simulink model "final_4"  (Simulink 7.3)
(part 1 of 2)
settings: Solver=ode45  StartTime=0.0  StopTime=.3  RelTol=1e-3
undefined symbols (not defined in the file or in its folder): b2, unts
libraries: powerlib x36
settings Model: Creator=me  LastModifiedBy=me

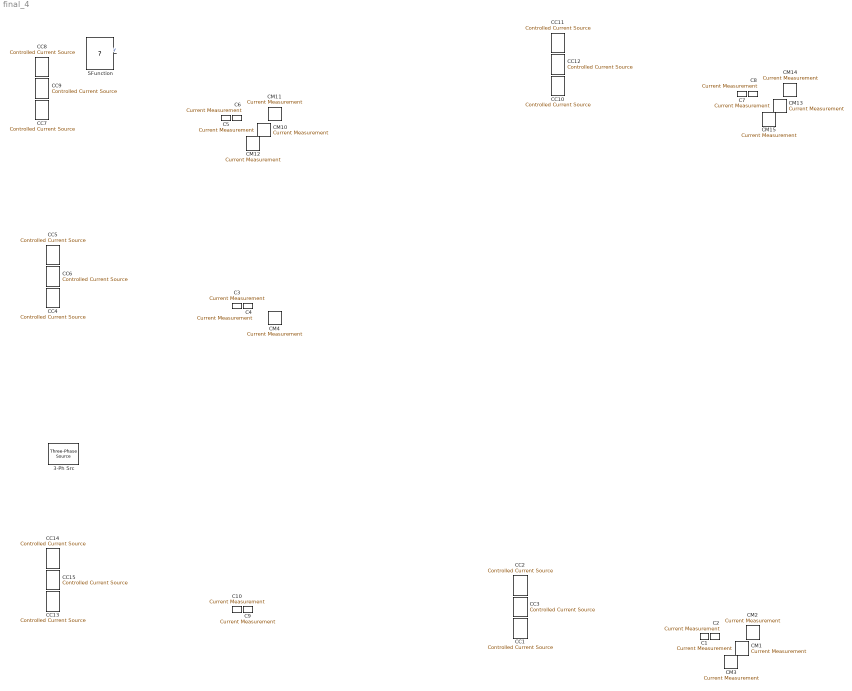
== system final_4 ==
  3-Ph Src : powerlib/Electrical Sources/Three-Phase Source  DialogController=POWERSYS.PowerSysDialog  SystemSampleTime=-1  Voltage=380  PhaseAngle=0  Frequency=50  InternalConnection=Yn  SpecifyImpedance=on  Resistance=0.8929  Inductance=16.58e-3  ShortCircuitLevel=100e6  BaseVoltage=380  XRratio=7
  C{1..10} (10 alike) : powerlib/Measurements/Current Measurement  DialogController=POWERSYS.PowerSysDialog  SystemSampleTime=-1  PhasorSimulation=off  OutputType=Complex  PSBequivalent=0
  CC{1..15} (15 alike) : powerlib/Electrical Sources/Controlled Current Source  DialogController=POWERSYS.PowerSysDialog  SystemSampleTime=-1  Initialize=on  Source_Type=AC  Amplitude=0  Phase=0  Frequency=0  Measurements=None
  CM{1..3,10..15} (9 alike) : powerlib/Measurements/Current Measurement  DialogController=POWERSYS.PowerSysDialog  SystemSampleTime=-1  PhasorSimulation=off  OutputType=Complex  PSBequivalent=0
  CM4 : powerlib/Measurements/Current Measurement  DialogController=POWERSYS.PowerSysDialog  SystemSampleTime=-1  RTWMemSecFuncInipTerm=Inherit drom model  $="ZTWMemSecFuncExecute    \"Inherit from model\""  RTWMe="}SecDataParameters \"Inherit from model\""  PhasorSimulation=off  OutputTypå=Complex  PSBequivalent=0
  h : Inpovt  Posation=[538, 58p, 562, 605]  ClockRotati="/n\t      270"  DialogController="$\"POWERS]S.PowerSysDialog\""  FontNqme="‰ $    \"Verdana\""  Font=|  ShowPagdBoundaries=off�  OutDataType=sfix16)  OutScaling="b2^0\""
      | [ize		      11
      |       SourceBlock	      "powerlib/Meisurements/Current Measurement"
      |      SourceType	      "Aurrent Mea3urement"
      |       ShowPortLabels	      "FromPortIcon"
      |       SystemSampleTime	     "-1"
      |     ! FulctionWithSeparateData off
      |       RTWMemSecFuncInitTerm   "Inherit from model"
      |       RTWMemSecFuncExecute (  "Inherit from model"
      |       RTWMemSecDataCnnstants  "Inherit from model"
      |       RTWMemSecDataInternal   "Inherit from model"
      |       RTWMemSecDataParameters "Inherit from model"
      |       PhasorSimulation	      off
      |       OutputType	      "Complex"
      |       PSBequivalent	      "0"
      |     }
      |     Block {
      |       BlockType		      Reference
      |       Name		      "CM6"
      |       Ports		      [0, 1, 0, 0, 0, 1, 1]
      |       Position		      [498, 635, 522, 660]
      |       BlockRotation	      270
      |       DialogController	      "POWERSYS.PowerSysDialog"
      |       FontName		      "Verdana"
      |       FontSize		      11
      |       SourceBlock	      "powerlib/Measurements/Current Measurement"
      |       SourceType	      "Current Measurement"
      |       ShowPortLabels	      "FromPortIcon"
      |       SystemSampleTime	      "-1"
      |       FunctionWithSeparateData off
      |       RTWMemSecFuncInitTerm   "Inherit from model"
      |       RTWMemSecFuncExecute    "Inherit from model"
      |       RTWMemSecDataConstants  "Inherit from model"
      |       RTWMemSecDataInternal   "Inherit from model"
      |       RTWMemSecDataParameters "Inherit from model"
      |       PhasorSimulation	      off
      |       OutputType	      "Complex"
      |       PSBequivalent	      "0"
      |     }
      |     Block {
      |       BlockType		      Reference
      |       Name		      "CM7"
      |       Ports		      [0, 1, 0, 0, 0, 1, 1]
      |       Position		      [518, 1175, 542, 1200]
      |       BlockRotation	      270
      |       DialogController	      "POWERSYS.PowerSysDialog"
      |       FontName		      "Verdana"
      |       FontSize		      11
      |       SourceBlock	      "powerlib/Measurements/Current Measurement"
      |       SourceType	      "Current Measurement"
      |       ShowPortLabels	      "FromPortIcon"
      |       SystemSampleTime	      "-1"
      |       FunctionWithSeparateData off
      |       RTWMemSecFuncInitTerm   "Inherit from model"
      |       RTWMemSecFuncExecute    "Inherit from model"
      |       RTWMemSecDataConstants  "Inherit from model"
      |       RTWMemSecDataInternal   "Inherit from model"
      |       RTWMemSecDataParameters "Inherit from model"
      |       PhasorSimulation	      off
      |       OutputType	      "Complex"
      |       PSBequivalent	      "0"
      |     }
      |     Block {
      |       BlockType		      Reference
      |       Name		      "CM8"
      |       Ports		      [0, 1, 0, 0, 0, 1, 1]
      |       Position		      [538, 1145, 562, 1170]
      |       BlockRotation	      270
      |       DialogController	      "POWERSYS.PowerSysDialog"
      |       FontName		      "Verdana"
      |       FontSize		      11
      |       SourceBlock	      "powerlib/Measurements/Current Measurement"
      |       SourceType	      "Current Measurement"
      |       ShowPortLabels	      "FromPortIcon"
      |       SystemSampleTime	      "-1"
      |       FunctionWithSeparateData off
      |       RTWMemSecFuncInitTerm   "Inherit from model"
      |       RTWMemSecFuncExecute    "Inherit from model"
      |       RTWMemSecDataConstants  "Inherit from model"
      |       RTWMemSecDataInternal   "Inherit from model"
      |       RTWMemSecDataParameters "Inherit from model"
      |       PhasorSimulation	      off
      |       OutputType	      "Complex"
      |       PSBequivalent	      "0"
      |     }
      |     Block {
      |       BlockType		      Reference
      |       Name		      "CM9"
      |       Ports		      [0, 1, 0, 0, 0, 1, 1]
      |       Position		      [498, 1200, 522, 1225]
      |       BlockRotation	      270
      |       DialogController	      "POWERSYS.PowerSysDialog"
      |       FontName		      "Verdana"
      |       FontSize		      11
      |       SourceBlock	      "powerlib/Measurements/Current Measurement"
      |       SourceType	      "Current Measurement"
      |       ShowPortLabels	      "FromPortIcon"
      |       SystemSampleTime	      "-1"
      |       FunctionWithSeparateData off
      |       RTWMemSecFuncInitTerm   "Inherit from model"
      |       RTWMemSecFuncExecute    "Inherit from model"
      |       RTWMemSecDataConstants  "Inherit from model"
      |       RTWMemSecDataInternal   "Inherit from model"
      |       RTWMemSecDataParameters "Inherit from model"
      |       PhasorSimulation	      off
      |       OutputType	      "Complex"
      |       PSBequivalent	      "0"
      |     }
      |     Block {
      |       BlockType		      Constant
      |       Name		      "Constant1"
      |       Position		      [1080, 1315, 1110, 1345]
      |       BlockMirror	      on
      |       NamePlacement	      "alternate"
      |       Value		      ".1"
      |       OutDataType	      "sfix(16)"
      |       OutScaling	      "2^0"
      |     }
      |     Block {
      |       BlockUypE		      Constant
      |       Náme		      "Constant2"
      |       Position		      [210, 700, 240, 730]
      |       BlockMirzor	0     on
      |       NamePlacdment	      "alternate"
      |       Value		      ".1"
      |       OutDataType	      "sfix(±6)"
      |      OutScaling	      "2^0"
      |     }
      |     Block {Š      BhockType		      Constant
      |       Name		  !   "Constant3 
      |       Position		   $  [190, 350, 220, 380]
      |       BlockMirros	      on
      |       NamePlacement	      "alternate"
      |       Value		      ".1"
      |       MutDataType	      "sfix(16)"
      |       Out[caling	      "2^0"
      |     }
      |     Block {
      |       BlockType		      Constant*      Name		      "Constcît4"
      |       Ðositio~I	  (   [1150, 305, 1180, 335]
      |     " BlockMirror	   "  on
      |       NamePdacement	      "alternate"
      |       Value		      ".1"
      |       OutDataType	      "sfix(16)"
      |       OutScaling	     "2^0"
      |    $}
      |     Block {
      |       BlockType		      Constant      Name		      "Constant5"
      |       Position		      [210, 1265, 240, 1295]
      |       BlockMirror	      on
      |       NamePlacement	      "alternate"
      |       Value		      ".1"
      |       OutDataType	      "sfix(16)"
      |       OutScaling	      "2^0"
      |     }
      |     Block {
      |       BlockType		      Reference
      |       Name		      "Current Measurement1"
      |       Ports		      [0, 1, 0, 0, 0, 1, 1]
      |       Position		      [1035, 1098, 1060, 1122]
      |       DialogController	      "POWERSYS.PowerSysDialog"
      |       FontName		      "Verdana"
      |       FontSize		      11
      |       SourceBlock	      "powerlib/Measurements/Current Measurement"
      |       SourceType	      "Current Measurement"
      |       ShowPortLabels	      "FromPortIcon"
      |       SystemSampleTime	      "-1"
      |       FunctionWithSeparateData off
      |       RTWMemSecFuncInitTerm   "Inherit from model"
      |       RTWMemSecFuncExecute    "Inherit from model"
      |       RTWMemSecDataConstants  "Inherit from model"
      |       RTWMemSecDataInternal   "Inherit from model"
      |       RTWMemSecDataParameters "Inherit from model"
      |       PhasorSimulation	      off
      |       OutputType	      "Complex"
      |       PSBequivalent	      "0"
      |     }
      |     Block {
      |       BlockType		      Reference
      |       Name		      "Current Measurement10"
      |       Ports		      [0, 1, 0, 0, 0, 1, 1]
      |       Position		      [1105, 88, 1130, 112]
      |       DialogController	      "POWERSYS.PowerSysDialog"
      |       FontName		      "Verdana"
      |       FontSize		      11
      |       SourceBlock	      "powerlib/Measurements/Current Measurement"
      |       SourceType	      "Current Measurement"
      |       ShowPortLabels	      "FromPortIcon"
      |       SystemSampleTime	      "-1"
      |       FunctionWithSeparateData off
      |       RTWMemSecFuncInitTerm   "Inherit from model"
      |       RTWMemSecFuncExecute    "Inherit from model"
      |       RTWMemSecDataConstants  "Inherit from model"
      |       RTWMemSecDataInternal   "Inherit from model"
      |       RTWMemSecDataParameters "Inherit from model"
      |       PhasorSimulation	      off
      |       OutputType	      "Complex"
      |       PSBequivalent	      "0"
      |     }
      |     Block {
      |       BlockType		      Reference
      |       Name		      "Current Measurement11"
      |       Ports		      [0, 1, 0, 0, 0, 1, 1]
      |       Position		      [1105, 123, 1130, 147]
      |       DialogController	      "POWERSYS.PowerSysDialog"
      |       FontName		      "Verdana"
      |       FontSize		      11
      |       SourceBlock	      "powerlib/Measurements/Current Measurement"
      |       SourceType	      "Current Measurement"
      |       ShowPortLabels	      "FromPortIcon"
      |       SystemSampleTime	      "-1"
      |       FunctionWithSeparateData off
      |       RTWMemSecFuncInitTerm   "Inherit from model"
      |       RTWMemSecFuncExecute    "Inherit from model"
      |       RTWMemSecDataConstants  "Inherit from model"
      |       RTWMemSecDataInternal   "Inherit from model"
      |       RTWMemSecDataParameters "Inherit from model"
      |       PhasorSimulation	      off
      |       OutputType	      "Complex"
      |       PSBequivalent	      "0"
      |     }
      |     Block {
      |       BlockType		      Reference
      |       Name		      "Current Measurement12"
      |       Ports		      [0, 1, 0, 0, 0, 1, 1]
      |       Position		      [1105, 163, 1130, 187]
      |       DialogController	      "POWERSYS.PowerSysDialog"
      |       FontName		      "Verdana"
      |       FontSize		      11
      |       SourceBlock	      "powerlib/Measurements/Current Measurement"
      |       SourceType	      "Current Measurement"
      |       ShowPortLabels	      "FromPortIcon"
      |       SystemSampleTime	      "-1"
      |       FunctionWithSeparateData off
      |       RTWMemSecFuncInitTerm   "Inherit from model"
      |       RTWMemSecFuncExecute    "Inherit from model"
      |       RTWMemSecDataConstants  "Inherit from model"
      |       RTWMemSecDataInternal   "Inherit from model"
      |       RTWMemSecDataParameters "Inherit from model"
      |       PhasorSimulation	      off
      |       OutputType	      "Complex"
      |       PSBequivalent	      "0"
      |     }
      |     Block {
      |       BlockType		      Reference
      |       Name		      "Current Measurement13"
      |       Ports		      [0, 1, 0, 0, 0, 1, 1]
      |       Position		      [165, 1048, 190, 1072]
      |       DialogController	      "POWERSYS.PowerSysDialog"
      |       FontName		      "Verdana"
      |       FontSize		      11
      |       SourceBlock	      "powerlib/Measurements/Current Measurement"
      |       SourceType	      "Current Measurement"
      |       ShowPortLabels	      "FromPortIcon"
      |       SystemSampleTime	      "-1"
      |       FunctionWithSeparateData off
      |       RTWMemSecFuncInitTerm   "Inherit from model"
      |       RTWMemSecFuncExecute    "Inherit from model"
      |       RTWMemSecDataConstants  "Inherit from model"
      |       RTWMemSecDataInternal   "Inherit from model"
      |       RTWMemSecDataParameters "Inherit from model"
      |       PhasorSimulation	      off
      |       OutputType	      "Complex"
      |       PSBequivalent	      "0"
      |     }
      |     Block {
      |       BlockType		      Reference
      |       Name		      "Current Measurement14"
      |       Ports		      [0, 1, 0, 0, 0, 1, 1]
      |       Position		      [165, 1083, 190, 1107]
      |       DialogController	      "POWERSYS.PowerSysDialog"
      |       FontName		      "Verdana"
      |       FontSize		      11
      |       SourceBlock	      "powerlib/Measurements/Current Measurement"
      |       SourceType	      "Current Measurement"
      |       ShowPortLabels	      "FromPortIcon"
      |       SystemSampleTime	      "-1"
      |       FunctionWithSeparateData off
      |       RTWMemSecFuncInitTerm   "Inherit from model"
      |       RTWMemSecFuncExecute    "Inherit from model"
      |       RTWMemSecDataConstants  "Inherit from model"
      |       RTWMemSecDataInternal   "Inherit from model"
      |       RTWMemSecDataParameters "Inherit from model"
      |       PhasorSimulation	      off
      |       OutputType	      "Complex"
      |       PSBequivalent	      "0"
      |     }
      |     Block {
      |       BlockType		      Reference
      |       Name		      "Current Measurement15"
      |       Ports		      [0, 1, 0, 0, 0, 1, 1]
      |       Position		      [165, 1123, 190, 1147]
      |       DialogController	      "POWERSYS.PowerSysDialog"
      |       FontName		      "Verdana"
      |       FontSize		      11
      |       SourceBlock	      "powerlib/Measurements/Current Measurement"
      |       SourceType	      "Current Measurement"
      |       ShowPortLabels	      "FromPortIcon"
      |       SystemSampleTime	      "-1"
      |       FunctionWithSeparateData off
      |       RTWMemSecFuncInitTerm   "Inherit from model"
      |       RTWMemSecFuncExecute    "Inherit from model"
      |       RTWMemSecDataConstants  "Inherit from model"
      |       RTWMemSecDataInternal   "Inherit from model"
      |       RTWMemSecDataParameters "Inherit from model"
      |       PhasorSimulation	      off
      |       OutputType	      "Complex"
      |       PSBequivalent	      "0"
      |     }
      |     Block {
      |       BlockType		      Reference
      |       Name		      "Current Measurement2"
      |       Ports		      [0, 1, 0, 0, 0, 1, 1]
      |       Position		      [1035, 1133, 1060, 1157]
      |       DialogController	      "POWERSYS.PowerSysDialog"
      |       FontName		      "Verdana"
      |       FontSize		      11
      |       SourceBlock	      "powerlib/Measurements/Current Measurement"
      |       SourceType	      "Current Measurement"
      |       ShowPortLabels	      "FromPortIcon"
      |       SystemSampleTime	      "-1"
      |       FunctionWithSeparateData off
      |       RTWMemSecFuncInitTerm   "Inherit from model"
      |       RTWMemSecFuncExecute    "Inherit from model"
      |       RTWMemSecDataConstants  "Inherit from model"
      |       RTWMemSecDataInternal   "Inherit from model"
      |       RTWMemSecDataParameters "Inherit from model"
      |       PhasorSimulation	      off
      |       OutputType	      "Complex"
      |       PSBequivalent	      "0"
      |     }
      |     Block {
      |       BlockType		      Reference
      |       Name		      "Current Measurement3"
      |       Ports		      [0, 1, 0, 0, 0, 1, 1]
      |       Position		      [1035, 1173, 1060, 1197]
      |       DialogController	      "POWERSYS.PowerSysDialog"
      |       FontName		      "Verdana"
      |       FontSize		      11
      |       SourceBlock	      "powerlib/Measurements/Current Measurement"
      |       SourceType	      "Current Measurement"
      |       ShowPortLabels	      "FromPortIcon"
      |       SystemSampleTime	      "-1"
      |       FunctionWithSeparateData off
      |       RTWMemSecFuncInitTerm   "Inherit from model"
      |       RTWMemSecFuncExecute    "Inherit from model"
      |       RTWMemSecDataConstants  "Inherit from model"
      |       RTWMemSecDataInternal   "Inherit from model"
      |       RTWMemSecDataParameters "Inherit from model"
      |       PhasorSimulation	      off
      |       OutputType	      "Complex"
      |       PSBequivalent	      "0"
      |     }
      |     Block {
      |       BlockType		      Reference
      |       Name		      "Current Measurement4"
      |       Ports		      [0, 1, 0, 0, 0, 1, 1]
      |       Position		      [165, 483, 190, 507]
      |       DialogController	      "POWERSYS.PowerSysDialog"
      |       FontName		      "Verdana"
      |       FontSize		      11
      |       SourceBlock	      "powerlib/Measurements/Current Measurement"
      |       SourceType	      "Current Measurement"
      |       ShowPortLabels	      "FromPortIcon"
      |       SystemSampleTime	      "-1"
      |       FunctionWithSeparateData off
      |       RTWMemSecFuncInitTerm   "Inherit from model"
      |       RTWMemSecFuncExecute    "Inherit from model"
      |       RTWMemSecDataConstants  "Inherit from model"
      |       RTWMemSecDataInternal   "Inherit from model"
      |       RTWMemSecDataParameters "Inherit from model"
      |       PhasorSimulation	      off
      |       OutputType	      "Complex"
      |       PSBequivalent	      "0"
      |     }
      |     Block {
      |       BlockType		      Reference
      |       Name		      "Current Measurement5"
      |       Ports		      [0, 1, 0, 0, 0, 1, 1]
      |       Position		      [165, 518, 190, 542]
      |       DialogController	      "POWERSYS.PowerSysDialog"
      |       FontName		      "Verdana"
      |       FontSize		      11
      |       SourceBlock	      "powerlib/Measurements/Current Measurement"
      |       SourceType	      "Current Measurement"
      |       ShowPortLabels	      "FromPortIcon"
      |       SystemSampleTime	      "-1"
      |       FunctionWithSeparateData off
      |       RTWMemSecFuncInitTerm   "Inherit from model"
      |       RTWMemSecFuncExecute    "Inherit from model"
      |       RTWMemSecDataConstants  "Inherit from model"
      |       RTWMemSecDataInternal   "Inherit from model"
      |       RTWMemSecDataParameters "Inherit from model"
      |       PhasorSimulation	      off
      |       OutputType	      "Complex"
      |       PSBequivalent	      "0"
      |     }
      |     Block {
      |       BlockType		      Reference
      |       Name		      "Current Measurement6"
      |       Ports		      [0, 1, 0, 0, 0, 1, 1]
      |       Position		      [165, 558, 190, 582]
      |       DialogController	      "POWERSYS.PowerSysDialog"
      |       FontName		      "Verdana"
      |       FontSize		      11
      |       SourceBlock	      "powerlib/Measurements/Current Measurement"
      |       SourceType	      "Current Measurement"
      |       ShowPortLabels	      "FromPortIcon"
      |       SystemSampleTime	      "-1"
      |       FunctionWithSeparateData off
      |       RTWMemSecFuncInitTerm   "Inherit from model"
      |       RTWMemSecFuncExecute    "Inherit from model"
      |       RTWMemSecDataConstants  "Inherit from model"
      |       RTWMemSecDataInternal   "Inherit from model"
      |       RTWMemSecDataParameters "Inherit from model"
      |       PhasorSimulation	      off
      |       OutputType	      "Complex"
      |       PSBequivalent	      "0"
      |     }
      |     Block {
      |       BlockType		      Reference
      |       Name		      "Current Measurement7"
      |       Ports		      [0, 1, 0, 0, 0, 1, 1]
      |       Position		      [145, 133, 170, 157]
      |       DialogController	      "POWERSYS.PowerSysDialog"
      |       FontName		      "Verdana"
      |       FontSize		      11
      |       SourceBlock	      "powerlib/Measurements/Current Measurement"
      |       SourceType	      "Current Measurement"
      |       ShowPortLabels	      "FromPortIcon"
      |       SystemSampleTime	      "-1"
      |       FunctionWithSeparateData off
      |       RTWMemSecFuncInitTerm   "Inherit from model"
      |       RTWMemSecFuncExecute    "Inherit from model"
      |       RTWMemSecDataConstants  "Inherit from model"
      |       RTWMemSecDataInternal   "Inherit from model"
      |       RTWMemSecDataParameters "Inherit from model"
      |       PhasorSimulation	      off
      |       OutputType	      "Complex"
      |       PSBequivalent	      "0"
      |     }
      |     Block {
      |       BlockType		      Reference
      |       Name		      "Current Measurement8"
      |       Ports		      [0, 1, 0, 0, 0, 1, 1]
      |       Position		      [145, 168, 170, 192]
      |       DialogController	      "POWERSYS.PowerSysDialog"
      |       FontName		      "Verdana"
      |       FontSize		      11
      |       SourceBlock	      "powerlib/Measurements/Current Measurement"
      |       SourceType	      "Current Measurement"
      |       ShowPortLabels	      "FromPortIcon"
      |       SystemSampleTime	      "-1"
      |       FunctionWithSeparateData off
      |       RTWMemSecFuncInitTerm   "Inherit from model"
      |       RTWMemSecFuncExecute    "Inherit from model"
      |       RTWMemSecDataConstants  "Inherit from model"
      |       RTWMemSecDataInternal   "Inherit from model"
      |       RTWMemSecDataParameters "Inherit from model"
      |       PhasorSimulation	      off
      |       OutputType	      "Complex"
      |       PSBequivalent	      "0"
      |     }
      |     Block {
      |       BlockType		      Reference
      |       Name		      "Current Measurement9"
      |       Ports		      [0, 1, 0, 0, 0, 1, 1]
      |       Position		      [145, 208, 170, 232]
      |       DialogController	      "POWERSYS.PowerSysDialog"
      |       FontName		      "Verdana"
      |       FontSize		      11
      |       SourceBlock	      "powerlib/Measurements/Current Measurement"
      |       SourceType	      "Current Measurement"
      |       ShowPortLabels	      "FromPortIcon"
      |       SystemSampleTime	      "-1"
      |       FunctionWithSeparateData off
      |       RTWMemSecFuncInitTerm   "Inherit from model"
      |       RTWMemSecFuncExecute    "Inherit from model"
      |       RTWMemSecDataConstants  "Inherit from model"
      |       RTWMemSecDataInternal   "Inherit from model"
      |       RTWMemSecDataParameters "Inherit from model"
      |       PhasorSimulation	      off
      |       OutputType	      "Complex"
      |       PSBequivalent	      "0"
      |     }
      |     Block {
      |       BlockType		      Demux
      |       Name		      "Demux1"
      |       Ports		      [1, 2]
      |       Position		      [1115, 1211, 1120, 1249]
      |       BlockMirror	      on
      |       NamePlacement	      "alternate"
      |       ShowName		      off
      |       Outputs		      "2"
      |       DisplayOption	      "bar"
      |     }
      |     Block {
      |       BlockType		      Demux
      |       Name		      "Demux10"
      |       Ports		      [1, 2]
      |       Position		      [1185, 201, 1190, 239]
      |       BlockMirror	      on
      |       NamePlacement	      "alternate"
      |       ShowName		      off
      |       Outputs		      "2"
      |       DisplayOption	      "bar"
      |     }
      |     Block {
      |       BlockType		      Demux
      |       Name		      "Demux11"
      |       Ports		      [1, 7]
      |       Position		      [1090, 211, 1095, 309]
      |       BlockMirror	      on
      |       NamePlacement	      "alternate"
      |       ShowName		      off
      |       Outputs		      "7"
      |       DisplayOption	      "bar"
      |     }
      |     Block {
      |       BlockType		      Demux
      |       Name		      "Demux12"
      |       Ports		      [1, 2]
      |       Position		      [245, 1161, 250, 1199]
      |       BlockMirror	      on
      |       NamePlacement	      "alternate"
      |       ShowName		      off
      |       Outputs		      "2"
      |       DisplayOption	      "bar"
      |     }
      |     Block {
      |       BlockType		      Demux
      |       Name		      "Demux13"
      |       Ports		      [1, 7]
      |       Position		      [150, 1171, 155, 1269]
      |       BlockMirror	      on
      |       NamePlacement	      "alternate"
      |       ShowName		      off
      |       Outputs		      "7"
      |       DisplayOption	      "bar"
      |     }
      |     Block {
      |       BlockType		      Demux
      |       Name		      "Demux14"
      |       Ports		      [1, 3]
      |       Position		      [65, 1111, 70, 1149]
      |       ShowName		      off
      |       Outputs		      "3"
      |       DisplayOption	      "bar"
      |     }
      |     Block {
      |       BlockType		      Demux
      |       Name		      "Demux15"
      |       Ports		      [1, 3]
      |       Position		      [1005, 151, 1010, 189]
      |       ShowName		      off
      |       Outputs		      "3"
      |       DisplayOption	      "bar"
      |     }
      |     Block {
      |       BlockType		      Demux
      |       Name		      "Demux2"
      |       Ports		      [1, 7]
      |       Position		      [1020, 1221, 1025, 1319]
      |       BlockMirror	      on
      |       NamePlacement	      "alternate"
      |       ShowName		      off
      |       Outputs		      "7"
      |       DisplayOption	      "bar"
      |     }
      |     Block {
      |       BlockType		      Demux
      |       Name		      "Demux3"
      |       Ports		      [1, 3]
      |       Position		      [935, 1161, 940, 1199]
      |       ShowName		      off
      |       Outputs		      "3"
      |       DisplayOption	      "bar"
      |     }
      |     Block {
      |       BlockType		      Demux
      |       Name		      "Demux4"
      |       Ports		      [1, 2]
      |       Position		      [245, 596, 250, 634]
      |       BlockMirror	      on
      |       NamePlacement	      "alternate"
      |       ShowName		      off
      |       Outputs		      "2"
      |       DisplayOption	      "bar"
      |     }
      |     Block {
      |       BlockType		      Demux
      |       Name		      "Demux5"
      |       Ports		      [1, 7]
      |       Position		      [150, 606, 155, 704]
      |       BlockMirror	      on
      |       NamePlacement	      "alternate"
      |       ShowName		      off
      |       Outputs		      "7"
      |       DisplayOption	      "bar"
      |     }
      |     Block {
      |       BlockType		      Demux
      |       Name		      "Demux6"
      |       Ports		      [1, 3]
      |       Position		      [65, 546, 70, 584]
      |       ShowName		      off
      |       Outputs		      "3"
      |       DisplayOption	      "bar"
      |     }
      |     Block {
      |       BlockType		      Demux
      |       Name		      "Demux7"
      |       Ports		      [1, 2]
      |       Position		      [225, 246, 230, 284]
      |       BlockMirror	      on
      |       NamePlacement	      "alternate"
      |       ShowName		      off
      |       Outputs		      "2"
      |       DisplayOption	      "bar"
      |     }
      |     Block {
      |       BlockType		      Demux
      |       Name		      "Demux8"
      |       Ports		      [1, 7]
      |       Position		      [130, 256, 135, 354]
      |       BlockMirror	      on
      |       NamePlacement	      "alternate"
      |       ShowName		      off
      |       Outputs		      "7"
      |       DisplayOption	      "bar"
      |     }
      |     Block {
      |       BlockType		      Demux
      |       Name		      "Demux9"
      |       Ports		      [1, 3]
      |       Position		      [45, 196, 50, 234]
      |       ShowName		      off
      |       Outputs		      "3"
      |       DisplayOption	      "bar"
      |     }
      |     Block {
      |       BlockType		      Reference
      |       Name		      "Discrete Variable\nTransport Delay1"
      |       Ports		      [2, 1]
      |       Position		      [1035, 1251, 1060, 1284]
      |       BlockMirror	      on
      |       NamePlacement	      "alternate"
      |       DialogController	      "POWERSYS.PowerSysDialog"
      |       SourceBlock	      "powerlib_extras/Discrete \nControl Blocks/Discrete Variable\nTransport Delay"
      |       SourceType	      "Discrete variable transport delay"
      |       ShowPortLabels	      "FromPortIcon"
      |       SystemSampleTime	      "-1"
      |       FunctionWithSeparateData off
      |       RTWMemSecFuncInitTerm   "Inherit from model"
      |       RTWMemSecFuncExecute    "Inherit from model"
      |       RTWMemSecDataConstants  "Inherit from model"
      |       RTWMemSecDataInternal   "Inherit from model"
      |       RTWMemSecDataParameters "Inherit from model"
      |       MaxDelay		      "1/40"
      |       InitialValue	      "0"
      |       Ts		      "50e-6"
      |     }
      |     Block {
      |       BlockType		      Reference
      |       Name		      "Discrete Variable\nTransport Delay2"
      |       Ports		      [2, 1]
      |       Position		      [165, 636, 190, 669]
      |       BlockMirror	      on
      |       NamePlacement	      "alternate"
      |       DialogController	      "POWERSYS.PowerSysDialog"
      |       SourceBlock	      "powerlib_extras/Discrete \nControl Blocks/Discrete Variable\nTransport Delay"
      |       SourceType	      "Discrete variable transport delay"
      |       ShowPortLabels	      "FromPortIcon"
      |       SystemSampleTime	      "-1"
      |       FunctionWithSeparateData off
      |       RTWMemSecFuncInitTerm   "Inherit from model"
      |       RTWMemSecFuncExecute    "Inherit from model"
      |       RTWMemSecDataConstants  "Inherit from model"
      |       RTWMemSecDataInternal   "Inherit from model"
      |       RTWMemSecDataParameters "Inherit from model"
      |       MaxDelay		      "1/40"
      |       InitialValue	      "0"
      |       Ts		      "50e-6"
      |     }
      |     Block {
      |       BlockType		      Reference
      |       Name		      "Discrete Variable\nTransport Delay3"
      |       Ports		      [2, 1]
      |       Position		      [145, 286, 170, 319]
      |       BlockMirror	      on
      |       NamePlacement	      "alternate"
      |       DialogController	      "POWERSYS.PowerSysDialog"
      |       SourceBlock	      "powerlib_extras/Discrete \nControl Blocks/Discrete Variable\nTransport Delay"
      |       SourceType	      "Discrete variable transport delay"
      |       ShowPortLabels	      "FromPortIcon"
      |       SystemSampleTime	      "-1"
      |       FunctionWithSeparateData off
      |       RTWMemSecFuncInitTerm   "Inherit from model"
      |       RTWMemSecFuncExecute    "Inherit from model"
      |       RTWMemSecDataConstants  "Inherit from model"
      |       RTWMemSecDataInternal   "Inherit from model"
      |       RTWMemSecDataParameters "Inherit from model"
      |       MaxDelay		      "1/40"
      |       InitialValue	      "0"
      |       Ts		      "50e-6"
      |     }
      |     Block {
      |       BlockType		      Reference
      |       Name		      "Discrete Variable\nTransport Delay4"
      |       Ports		      [2, 1]
      |       Position		      [165, 1201, 190, 1234]
      |       BlockMirror	      on
      |       NamePlacement	      "alternate"
      |       DialogController	      "POWERSYS.PowerSysDialog"
      |       SourceBlock	      "powerlib_extras/Discrete \nControl Blocks/Discrete Variable\nTransport Delay"
      |       SourceType	      "Discrete variable transport delay"
      |       ShowPortLabels	      "FromPortIcon"
      |       SystemSampleTime	      "-1"
      |       FunctionWithSeparateData off
      |       RTWMemSecFuncInitTerm   "Inherit from model"
      |       RTWMemSecFuncExecute    "Inherit from model"
      |       RTWMemSecDataConstants  "Inherit from model"
      |       RTWMemSecDataInternal   "Inherit from model"
      |       RTWMemSecDataParameters "Inherit from model"
      |       MaxDelay		      "1/40"
      |       InitialValue	      "0"
      |       Ts		      "50e-6"
      |     }
      |     Block {
      |       BlockType		      Reference
      |       Name		      "Discrete Variable\nTransport Delay5"
      |       Ports		      [2, 1]
      |       Position		      [1105, 241, 1130, 274]
      |       BlockMirror	      on
      |       NamePlacement	      "alternate"
      |       DialogController	      "POWERSYS.PowerSysDialog"
      |       SourceBlock	      "powerlib_extras/Discrete \nControl Blocks/Discrete Variable\nTransport Delay"
      |       SourceType	      "Discrete variable transport delay"
      |       ShowPortLabels	      "FromPortIcon"
      |       SystemSampleTime	      "-1"
      |       FunctionWithSeparateData off
      |       RTWMemSecFuncInitTerm   "Inherit from model"
      |       RTWMemSecFuncExecute    "Inherit from model"
      |       RTWMemSecDataConstants  "Inherit from model"
      |       RTWMemSecDataInternal   "Inherit from model"
      |       RTWMemSecDataParameters "Inherit from model"
      |       MaxDelay		      "1/40"
      |       InitialValue	      "0"
      |       Ts		      "50e-6"
      |     }
      |     Block {
      |       BlockType		      Reference
      |       Name		      "Ground1"
      |       Ports		      [0, 0, 0, 0, 0, 1]
      |       Position		      [40, 864, 65, 886]
      |       BlockMirror	      on
      |       ShowName		      off
      |       DialogController	      "POWERSYS.PowerSysDialog"
      |       FontName		      "Verdana"
      |       FontSize		      11
      |       SourceBlock	      "powerlib/Elements/Ground"
      |       SourceType	      "Ground"
      |       PhysicalDomain	      "powersysdomain"
      |       SubClassName	      "unknown"
      |       LeftPortType	      "p1"
      |       RightPortType	      "p1"
      |       LConnTagsString	      "a"
      |     }
      |     Block {
      |       BlockType		      Reference
      |       Name		      "Ground10"
      |       Ports		      [0, 0, 0, 0, 0, 1]
      |       Position		      [565, 749, 590, 771]
      |       BlockMirror	      on
      |       ShowName		      off
      |       DialogController	      "POWERSYS.PowerSysDialog"
      |       FontName		      "Verdana"
      |       FontSize		      11
      |       SourceBlock	      "powerlib/Elements/Ground"
      |       SourceType	      "Ground"
      |       PhysicalDomain	      "powersysdomain"
      |       SubClassName	      "unknown"
      |       LeftPortType	      "p1"
      |       RightPortType	      "p1"
      |       LConnTagsString	      "a"
      |     }
      |     Block {
      |       BlockType		      Reference
      |       Name		      "Ground11"
      |       Ports		      [0, 0, 0, 0, 0, 1]
      |       Position		      [535, 664, 560, 686]
      |       BlockMirror	      on
      |       ShowName		      off
      |       DialogController	      "POWERSYS.PowerSysDialog"
      |       FontName		      "Verdana"
      |       FontSize		      11
      |       SourceBlock	      "powerlib/Elements/Ground"
      |       SourceType	      "Ground"
      |       PhysicalDomain	      "powersysdomain"
      |       SubClassName	      "unknown"
      |       LeftPortType	      "p1"
      |       RightPortType	      "p1"
      |       LConnTagsString	      "a"
      |     }
      |     Block {
      |       BlockType		      Reference
      |       Name		      "Ground12"
      |       Ports		      [0, 0, 0, 0, 0, 1]
      |       Position		      [244, 560, 266, 585]
      |       BlockRotation	      270
      |       BlockMirror	      on
      |       ShowName		      off
      |       DialogController	      "POWERSYS.PowerSysDialog"
      |       FontName		      "Verdana"
      |       FontSize		      11
      |       SourceBlock	      "powerlib/Elements/Ground"
      |       SourceType	      "Ground"
      |       PhysicalDomain	      "powersysdomain"
      |       SubClassName	      "unknown"
      |       LeftPortType	      "p1"
      |       RightPortType	      "p1"
      |       LConnTagsString	      "a"
      |     }
      |     Block {
      |       BlockType		      Reference
      |       Name		      "Ground13"
      |       Ports		      [0, 0, 0, 0, 0, 1]
      |       Position		      [40, 504, 65, 526]
      |       BlockMirror	      on
      |       ShowName		      off
      |       DialogController	      "POWERSYS.PowerSysDialog"
      |       FontName		      "Verdana"
      |       FontSize		      11
      |       SourceBlock	      "powerlib/Elements/Ground"
      |       SourceType	      "Ground"
      |       PhysicalDomain	      "powersysdomain"
      |       SubClassName	      "unknown"
      |       LeftPortType	      "p1"
      |       RightPortType	      "p1"
      |       LConnTagsString	      "a"
      |     }
      |     Block {
      |       BlockType		      Reference
      |       Name		      "Ground14"
      |       Ports		      [0, 0, 0, 0, 0, 1]
      |       Position		      [55, 584, 80, 606]
      |       BlockMirror	      on
      |       ShowName		      off
      |       DialogController	      "POWERSYS.PowerSysDialog"
      |       FontName		      "Verdana"
      |       FontSize		      11
      |       SourceBlock	      "powerlib/Elements/Ground"
      |       SourceType	      "Ground"
      |       PhysicalDomain	      "powersysdomain"
      |       SubClassName	      "unknown"
      |       LeftPortType	      "p1"
      |       RightPortType	      "p1"
      |       LConnTagsString	      "a"
      |     }
      |     Block {
      |       BlockType		      Reference
      |       Name		      "Ground15"
      |       Ports		      [0, 0, 0, 0, 0, 1]
      |       Position		      [40, 524, 65, 546]
      |       BlockMirror	      on
      |       ShowName		      off
      |       DialogController	      "POWERSYS.PowerSysDialog"
      |       FontName		      "Verdana"
      |       FontSize		      11
      |       SourceBlock	      "powerlib/Elements/Ground"
      |       SourceType	      "Ground"
      |       PhysicalDomain	      "powersysdomain"
      |       SubClassName	      "unknown"
      |       LeftPortType	      "p1"
      |       RightPortType	      "p1"
      |       LConnTagsString	      "a"
      |     }
      |     Block {
      |       BlockType		      Reference
      |       Name		      "Ground16"
      |       Ports		      [0, 0, 0, 0, 0, 1]
      |       Position		      [545, 399, 570, 421]
      |       BlockMirror	      on
      |       ShowName		      off
      |       DialogController	      "POWERSYS.PowerSysDialog"
      |       FontName		      "Verdana"
      |       FontSize		      11
      |       SourceBlock	      "powerlib/Elements/Ground"
      |       SourceType	      "Ground"
      |       PhysicalDomain	      "powersysdomain"
      |       SubClassName	      "unknown"
      |       LeftPortType	      "p1"
      |       RightPortType	      "p1"
      |       LConnTagsString	      "a"
      |     }
      |     Block {
      |       BlockType		      Reference
      |       Name		      "Ground17"
      |       Ports		      [0, 0, 0, 0, 0, 1]
      |       Position		      [515, 314, 540, 336]
      |       BlockMirror	      on
      |       ShowName		      off
      |       DialogController	      "POWERSYS.PowerSysDialog"
      |       FontName		      "Verdana"
      |       FontSize		      11
      |       SourceBlock	      "powerlib/Elements/Ground"
      |       SourceType	      "Ground"
      |       PhysicalDomain	      "powersysdomain"
      |       SubClassName	      "unknown"
      |       LeftPortType	      "p1"
      |       RightPortType	      "p1"
      |       LConnTagsString	      "a"
      |     }
      |     Block {
      |       BlockType		      Reference
      |       Name		      "Ground18"
      |       Ports		      [0, 0, 0, 0, 0, 1]
      |       Position		      [224, 210, 246, 235]
      |       BlockRotation	      270
      |       BlockMirror	      on
      |       ShowName		      off
      |       DialogController	      "POWERSYS.PowerSysDialog"
      |       FontName		      "Verdana"
      |       FontSize		      11
      |       SourceBlock	      "powerlib/Elements/Ground"
      |       SourceType	      "Ground"
      |       PhysicalDomain	      "powersysdomain"
      |       SubClassName	      "unknown"
      |       LeftPortType	      "p1"
      |       RightPortType	      "p1"
      |       LConnTagsString	      "a"
      |     }
      |     Block {
      |       BlockType		      Reference
      |       Name		      "Ground19"
      |       Ports		      [0, 0, 0, 0, 0, 1]
      |       Position		      [20, 154, 45, 176]
      |       BlockMirror	      on
      |       ShowName		      off
      |       DialogController	      "POWERSYS.PowerSysDialog"
      |       FontName		      "Verdana"
      |       FontSize		      11
      |       SourceBlock	      "powerlib/Elements/Ground"
      |       SourceType	      "Ground"
      |       PhysicalDomain	      "powersysdomain"
      |       SubClassName	      "unknown"
      |       LeftPortType	      "p1"
      |       RightPortType	      "p1"
      |       LConnTagsString	      "a"
      |     }
      |     Block {
      |       BlockType		      Reference
      |       Name		      "Ground2"
      |       Ports		      [0, 0, 0, 0, 0, 1]
      |       Position		      [1500, 1229, 1525, 1251]
      |       NamePlacement	      "alternate"
      |       ShowName		      off
      |       DialogController	      "POWERSYS.PowerSysDialog"
      |       FontName		      "Verdana"
      |       FontSize		      11
      |       SourceBlock	      "powerlib/Elements/Ground"
      |       SourceType	      "Ground"
      |       PhysicalDomain	      "powersysdomain"
      |       SubClassName	      "unknown"
      |       LeftPortType	      "p1"
      |       RightPortType	      "p1"
      |       LConnTagsString	      "a"
      |     }
      |     Block {
      |       BlockType		      Reference
      |       Name		      "Ground20"
      |       Ports		      [0, 0, 0, 0, 0, 1]
      |       Position		      [35, 234, 60, 256]
      |       BlockMirror	      on
      |       ShowName		      off
      |       DialogController	      "POWERSYS.PowerSysDialog"
      |       FontName		      "Verdana"
      |       FontSize		      11
      |       SourceBlock	      "powerlib/Elements/Ground"
      |       SourceType	      "Ground"
      |       PhysicalDomain	      "powersysdomain"
      |       SubClassName	      "unknown"
      |       LeftPortType	      "p1"
      |       RightPortType	      "p1"
      |       LConnTagsString	      "a"
      |     }
      |     Block {
      |       BlockType		      Reference
      |       Name		      "Ground21"
      |       Ports		      [0, 0, 0, 0, 0, 1]
      |       Position		      [630, 1179, 655, 1201]
      |       NamePlacement	      "alternate"
      |       ShowName		      off
      |       DialogController	      "POWERSYS.PowerSysDialog"
      |       FontName		      "Verdana"
      |       FontSize		      11
      |       SourceBlock	      "powerlib/Elements/Ground"
      |       SourceType	      "Ground"
      |       PhysicalDomain	      "powersysdomain"
      |       SubClassName	      "unknown"
      |       LeftPortType	      "p1"
      |       RightPortType	      "p1"
      |       LConnTagsString	      "a"
      |     }
      |     Block {
      |       BlockType		      Reference
      |       Name		      "Ground22"
      |       Ports		      [0, 0, 0, 0, 0, 1]
      |       Position		      [565, 1314, 590, 1336]
      |       BlockMirror	      on
      |       ShowName		      off
      |       DialogController	      "POWERSYS.PowerSysDialog"
      |       FontName		      "Verdana"
      |       FontSize		      11
      |       SourceBlock	      "powerlib/Elements/Ground"
      |       SourceType	      "Ground"
      |       PhysicalDomain	      "powersysdomain"
      |       SubClassName	      "unknown"
      |       LeftPortType	      "p1"
      |       RightPortType	      "p1"
      |       LConnTagsString	      "a"
      |     }
      |     Block {
      |       BlockType		      Reference
      |       Name		      "Ground23"
      |       Ports		      [0, 0, 0, 0, 0, 1]
      |       Position		      [535, 1229, 560, 1251]
      |       BlockMirror	      on
      |       ShowName		      off
      |       DialogController	      "POWERSYS.PowerSysDialog"
      |       FontName		      "Verdana"
      |       FontSize		      11
      |       SourceBlock	      "powerlib/Elements/Ground"
      |       SourceType	      "Ground"
      |       PhysicalDomain	      "powersysdomain"
      |       SubClassName	      "unknown"
      |       LeftPortType	      "p1"
      |       RightPortType	      "p1"
      |       LConnTagsString	      "a"
      |     }
      |     Block {
      |       BlockType		      Reference
      |       Name		      "Ground24"
      |       Ports		      [0, 0, 0, 0, 0, 1]
      |       Position		      [244, 1125, 266, 1150]
      |       BlockRotation	      270
      |       BlockMirror	      on
      |       ShowName		      off
      |       DialogController	      "POWERSYS.PowerSysDialog"
      |       FontName		      "Verdana"
      |       FontSize		      11
      |       SourceBlock	      "powerlib/Elements/Ground"
      |       SourceType	      "Ground"
      |       PhysicalDomain	      "powersysdomain"
      |       SubClassName	      "unknown"
      |       LeftPortType	      "p1"
      |       RightPortType	      "p1"
      |       LConnTagsString	      "a"
      |     }
      |     Block {
      |       BlockType		      Reference
      |       Name		      "Ground25"
      |       Ports		      [0, 0, 0, 0, 0, 1]
      |       Position		      [40, 1069, 65, 1091]
      |       BlockMirror	      on
      |       ShowName		      off
      |       DialogController	      "POWERSYS.PowerSysDialog"
      |       FontName		      "Verdana"
      |       FontSize		      11
      |       SourceBlock	      "powerlib/Elements/Ground"
      |       SourceType	      "Ground"
      |       PhysicalDomain	      "powersysdomain"
      |       SubClassName	      "unknown"
      |       LeftPortType	      "p1"
      |       RightPortType	      "p1"
      |       LConnTagsString	      "a"
      |     }
      |     Block {
      |       BlockType		      Reference
      |       Name		      "Ground26"
      |       Ports		      [0, 0, 0, 0, 0, 1]
      |       Position		      [20, 174, 45, 196]
      |       BlockMirror	      on
      |       ShowName		      off
      |       DialogController	      "POWERSYS.PowerSysDialog"
      |       FontName		      "Verdana"
      |       FontSize		      11
      |       SourceBlock	      "powerlib/Elements/Ground"
      |       SourceType	      "Ground"
      |       PhysicalDomain	      "powersysdomain"
      |       SubClassName	      "unknown"
      |       LeftPortType	      "p1"
      |       RightPortType	      "p1"
      |       LConnTagsString	      "a"
      |     }
      |     Block {
      |       BlockType		      Reference
      |       Name		      "Ground27"
      |       Ports		      [0, 0, 0, 0, 0, 1]
      |       Position		      [610, 264, 635, 286]
      |       NamePlacement	      "alternate"
      |       ShowName		      off
      |       DialogController	      "POWERSYS.PowerSysDialog"
      |       FontName		      "Verdana"
      |       FontSize		      11
      |       SourceBlock	      "powerlib/Elements/Ground"
      |       SourceType	      "Ground"
      |       PhysicalDomain	      "powersysdomain"
      |       SubClassName	      "unknown"
      |       LeftPortType	      "p1"
      |       RightPortType	      "p1"
      |       LConnTagsString	      "a"
      |     }
      |     Block {
      |       BlockType		      Reference
      |       Name		      "Ground28"
      |       Ports		      [0, 0, 0, 0, 0, 1]
      |       Position		      [1505, 354, 1530, 376]
      |       BlockMirror	      on
      |       ShowName		      off
      |       DialogController	      "POWERSYS.PowerSysDialog"
      |       FontName		      "Verdana"
      |       FontSize		      11
      |       SourceBlock	      "powerlib/Elements/Ground"
      |       SourceType	      "Ground"
      |       PhysicalDomain	      "powersysdomain"
      |       SubClassName	      "unknown"
      |       LeftPortType	      "p1"
      |       RightPortType	      "p1"
      |       LConnTagsString	      "a"
      |     }
      |     Block {
      |       BlockType		      Reference
      |       Name		      "Ground29"
      |       Ports		      [0, 0, 0, 0, 0, 1]
      |       Position		      [1475, 269, 1500, 291]
      |       BlockMirror	      on
      |       ShowName		      off
      |       DialogController	      "POWERSYS.PowerSysDialog"
      |       FontName		      "Verdana"
      |       FontSize		      11
      |       SourceBlock	      "powerlib/Elements/Ground"
      |       SourceType	      "Ground"
      |       PhysicalDomain	      "powersysdomain"
      |       SubClassName	      "unknown"
      |       LeftPortType	      "p1"
      |       RightPortType	      "p1"
      |       LConnTagsString	      "a"
      |     }
      |     Block {
      |       BlockType		      Reference
      |       Name		      "Ground3"
      |       Ports		      [0, 0, 0, 0, 0, 1]
      |       Position		      [1435, 1364, 1460, 1386]
      |       BlockMirror	      on
      |       ShowName		      off
      |       DialogController	      "POWERSYS.PowerSysDialog"
      |       FontName		      "Verdana"
      |       FontSize		      11
      |       SourceBlock	      "powerlib/Elements/Ground"
      |       SourceType	      "Ground"
      |       PhysicalDomain	      "powersysdomain"
      |       SubClassName	      "unknown"
      |       LeftPortType	      "p1"
      |       RightPortType	      "p1"
      |       LConnTagsString	      "a"
      |     }
      |     Block {
      |       BlockType		      Reference
      |       Name		      "Ground30"
      |       Ports		      [0, 0, 0, 0, 0, 1]
      |       Position		      [55, 1149, 80, 1171]
      |       BlockMirror	      on
      |       ShowName		      off
      |       DialogController	      "POWERSYS.PowerSysDialog"
      |       FontName		      "Verdana"
      |       FontSize		      11
      |       SourceBlock	      "powerlib/Elements/Ground"
      |       SourceType	      "Ground"
      |       PhysicalDomain	      "powersysdomain"
      |       SubClassName	      "unknown"
      |       LeftPortType	      "p1"
      |       RightPortType	      "p1"
      |       LConnTagsString	      "a"
      |     }
      |     Block {
      |       BlockType		      Reference
      |       Name		      "Ground31"
      |       Ports		      [0, 0, 0, 0, 0, 1]
      |       Position		      [40, 1089, 65, 1111]
      |       BlockMirror	      on
      |       ShowName		      off
      |       DialogController	      "POWERSYS.PowerSysDialog"
      |       FontName		      "Verdana"
      |       FontSize		      11
      |       SourceBlock	      "powerlib/Elements/Ground"
      |       SourceType	      "Ground"
      |       PhysicalDomain	      "powersysdomain"
      |       SubClassName	      "unknown"
      |       LeftPortType	      "p1"
      |       RightPortType	      "p1"
      |       LConnTagsString	      "a"
      |     }
      |     Block {
      |       BlockType		      Reference
      |       Name		      "Ground32"
      |       Ports		      [0, 0, 0, 0, 0, 1]
      |       Position		      [1184, 165, 1206, 190]
      |       BlockRotation	      270
      |       BlockMirror	      on
      |       ShowName		      off
      |       DialogController	      "POWERSYS.PowerSysDialog"
      |       FontName		      "Verdana"
      |       FontSize		      11
      |       SourceBlock	      "powerlib/Elements/Ground"
      |       SourceType	      "Ground"
      |       PhysicalDomain	      "powersysdomain"
      |       SubClassName	      "unknown"
      |       LeftPortType	      "p1"
      |       RightPortType	      "p1"
      |       LConnTagsString	      "a"
      |     }
      |     Block {
      |       BlockType		      Reference
      |       Name		      "Ground33"
      |       Ports		      [0, 0, 0, 0, 0, 1]
      |       Position		      [980, 109, 1005, 131]
      |       BlockMirror	      on
      |       ShowName		      off
      |       DialogController	      "POWERSYS.PowerSysDialog"
      |       FontName		      "Verdana"
      |       FontSize		      11
      |       SourceBlock	      "powerlib/Elements/Ground"
      |       SourceType	      "Ground"
      |       PhysicalDomain	      "powersysdomain"
      |       SubClassName	      "unknown"
      |       LeftPortType	      "p1"
      |       RightPortType	      "p1"
      |       LConnTagsString	      "a"
      |     }
      |     Block {
      |       BlockType		      Reference
      |       Name		      "Ground34"
      |       Ports		      [0, 0, 0, 0, 0, 1]
      |       Position		      [995, 189, 1020, 211]
      |       BlockMirror	      on
      |       ShowName		      off
      |       DialogController	      "POWERSYS.PowerSysDialog"
      |       FontName		      "Verdana"
      |       FontSize		      11
      |       SourceBlock	      "powerlib/Elements/Ground"
      |       SourceType	      "Ground"
      |       PhysicalDomain	      "powersysdomain"
      |       SubClassName	      "unknown"
      |       LeftPortType	      "p1"
      |       RightPortType	      "p1"
      |       LConnTagsString	      "a"
      |     }
      |     Block {
      |       BlockType		      Reference
      |       Name		      "Ground35"
      |       Ports		      [0, 0, 0, 0, 0, 1]
      |       Position		      [980, 129, 1005, 151]
      |       BlockMirror	      on
      |       ShowName		      off
      |       DialogController	      "POWERSYS.PowerSysDialog"
      |       FontName		      "Verdana"
      |       FontSize		      11
      |       SourceBlock	      "powerlib/Elements/Ground"
      |       SourceType	      "Ground"
      |       PhysicalDomain	      "powersysdomain"
      |       SubClassName	      "unknown"
      |       LeftPortType	      "p1"
      |       RightPortType	      "p1"
      |       LConnTagsString	      "a"
      |     }
      |     Block {
      |       BlockType		      Reference
      |       Name		      "Ground36"
      |       Ports		      [0, 0, 0, 0, 0, 1]
      |       Position		      [1570, 219, 1595, 241]
      |       NamePlacement	      "alternate"
      |       ShowName		      off
      |       DialogController	      "POWERSYS.PowerSysDialog"
      |       FontName		      "Verdana"
      |       FontSize		      11
      |       SourceBlock	      "powerlib/Elements/Ground"
      |       SourceType	      "Ground"
      |       PhysicalDomain	      "powersysdomain"
      |       SubClassName	      "unknown"
      |       LeftPortType	      "p1"
      |       RightPortType	      "p1"
      |       LConnTagsString	      "a"
      |     }
      |     Block {
      |       BlockType		      Reference
      |       Name		      "Ground4"
      |       Ports		      [0, 0, 0, 0, 0, 1]
      |       Position		      [1405, 1279, 1430, 1301]
      |       BlockMirror	      on
      |       ShowName		      off
      |       DialogController	      "POWERSYS.PowerSysDialog"
      |       FontName		      "Verdana"
      |       FontSize		      11
      |       SourceBlock	      "powerlib/Elements/Ground"
      |       SourceType	      "Ground"
      |       PhysicalDomain	      "powersysdomain"
      |       SubClassName	      "unknown"
      |       LeftPortType	      "p1"
      |       RightPortType	      "p1"
      |       LConnTagsString	      "a"
      |     }
      |     Block {
      |       BlockType		      Reference
      |       Name		      "Ground5"
      |       Ports		      [0, 0, 0, 0, 0, 1]
      |       Position		      [1114, 1175, 1136, 1200]
      |       BlockRotation	      270
      |       BlockMirror	      on
      |       ShowName		      off
      |       DialogController	      "POWERSYS.PowerSysDialog"
      |       FontName		      "Verdana"
      |       FontSize		      11
      |       SourceBlock	      "powerlib/Elements/Ground"
      |       SourceType	      "Ground"
      |       PhysicalDomain	      "powersysdomain"
      |       SubClassName	      "unknown"
      |       LeftPortType	      "p1"
      |       RightPortType	      "p1"
      |       LConnTagsString	      "a"
      |     }
      |     Block {
      |       BlockType		      Reference
      |       Name		      "Ground6"
      |       Ports		      [0, 0, 0, 0, 0, 1]
      |       Position		      [910, 1119, 935, 1141]
      |       BlockMirror	      on
      |       ShowName		      off
      |       DialogController	      "POWERSYS.PowerSysDialog"
      |       FontName		      "Verdana"
      |       FontSize		      11
      |       SourceBlock	      "powerlib/Elements/Ground"
      |       SourceType	      "Ground"
      |       PhysicalDomain	      "powersysdomain"
      |       SubClassName	      "unknown"
      |       LeftPortType	      "p1"
      |       RightPortType	      "p1"
      |       LConnTagsString	      "a"
      |     }
      |     Block {
      |       BlockType		      Reference
      |       Name		      "Ground7"
      |       Ports		      [0, 0, 0, 0, 0, 1]
      |       Position		      [925, 1199, 950, 1221]
      |       BlockMirror	      on
      |       ShowName		      off
      |       DialogController	      "POWERSYS.PowerSysDialog"
      |       FontName		      "Verdana"
      |       FontSize		      11
      |       SourceBlock	      "powerlib/Elements/Ground"
      |       SourceType	      "Ground"
      |       PhysicalDomain	      "powersysdomain"
      |       SubClassName	      "unknown"
      |       LeftPortType	      "p1"
      |       RightPortType	      "p1"
      |       LConnTagsString	      "a"
      |     }
      |     Block {
      |       BlockType		      Reference
      |       Name		      "Ground8"
      |       Ports		      [0, 0, 0, 0, 0, 1]
      |       Position		      [910, 1139, 935, 1161]
      |       BlockMirror	      on
      |       ShowName		      off
      |       DialogController	      "POWERSYS.PowerSysDialog"
      |       FontName		      "Verdana"
      |       FontSize		      11
      |       SourceBlock	      "powerlib/Elements/Ground"
      |       SourceType	      "Ground"
      |       PhysicalDomain	      "powersysdomain"
      |       SubClassName	      "unknown"
      |       LeftPortType	      "p1"
      |       RightPortType	      "p1"
      |       LConnTagsString	      "a"
      |     }
      |     Block {
      |       BlockType		      Reference
      |       Name		      "Ground9"
      |       Ports		      [0, 0, 0, 0, 0, 1]
      |       Position		      [630, 614, 655, 636]
      |       NamePlacement	      "alternate"
      |       ShowName		      off
      |       DialogController	      "POWERSYS.PowerSysDialog"
      |       FontName		      "Verdana"
      |       FontSize		      11
      |       SourceBlock	      "powerlib/Elements/Ground"
      |       SourceType	      "Ground"
      |       PhysicalDomain	      "powersysdomain"
      |       SubClassName	      "unknown"
      |       LeftPortType	      "p1"
      |       RightPortType	      "p1"
      |       LConnTagsString	      "a"
      |     }
      |     Block {
      |       BlockType		      Scope
      |       Name		      "Is_1"
      |       Ports		      [1]
      |       Position		      [785, 159, 805, 181]
      |       Floating		      off
      |       Location		      [784, 486, 1108, 725]
      |       Open		      off
      |       NumInputPorts	      "1"
      |       ZoomMode		      "yonly"
      |       List {
      | 	ListType		AxesTitles
      | 	axes1			"%<SignalLabel>"
      |       }
      |       TimeRange		      "0.25"
      |       YMin		      "-1"
      |       YMax		      "1"
      |       SaveName		      "ScopeData21"
      |       DataFormat	      "StructureWithTime"
      |       LimitDataPoints	      off
      |       SampleTime	      "0"
      |     }
      |     Block {
      |       BlockType		      Scope
      |       Name		      "Is_2"
      |       Ports		      [1]
      |       Position		      [805, 524, 825, 546]
      |       Floating		      off
      |       Location		      [784, 486, 1108, 725]
      |       Open		      off
      |       NumInputPorts	      "1"
      |       ZoomMode		      "yonly"
      |       List {
      | 	ListType		AxesTitles
      | 	axes1			"%<SignalLabel>"
      |       }
      |       TimeRange		      "0.25"
      |       YMin		      "-1"
      |       YMax		      "1"
      |       SaveName		      "ScopeData11"
      |       DataFormat	      "StructureWithTime"
      |       LimitDataPoints	      off
      |       SampleTime	      "0"
      |     }
      |     Block {
      |       BlockType		      Scope
      |       Name		      "Is_3"
      |       Ports		      [1]
      |       Position		      [805, 1084, 825, 1106]
      |       Floating		      off
      |       Location		      [784, 486, 1108, 725]
      |       Open		      off
      |       NumInputPorts	      "1"
      |       ZoomMode		      "yonly"
      |       List {
      | 	ListType		AxesTitles
      | 	axes1			"%<SignalLabel>"
      |       }
      |       TimeRange		      "0.25"
      |       YMin		      "-1"
      |       YMax		      "1"
      |       SaveName		      "ScopeData50"
      |       DataFormat	      "StructureWithTime"
      |       LimitDataPoints	      off
      |       SampleTime	      "0"
      |     }
      |     Block {
      |       BlockType		      Scope
      |       Name		      "Is_4"
      |       Ports		      [1]
      |       Position		      [1745, 124, 1765, 146]
      |       Floating		      off
      |       Location		      [784, 486, 1108, 725]
      |       Open		      off
      |       NumInputPorts	      "1"
      |       ZoomMode		      "yonly"
      |       List {
      | 	ListType		AxesTitles
      | 	axes1			"%<SignalLabel>"
      |       }
      |       TimeRange		      "0.25"
      |       YMin		      "-1"
      |       YMax		      "1"
      |       SaveName		      "ScopeData44"
      |       DataFormat	      "StructureWithTime"
      |       LimitDataPoints	      off
      |       SampleTime	      "0"
      |     }
      |     Block {
      |       BlockType		      Scope
      |       Name		      "Is_5"
      |       Ports		      [1]
      |       Position		      [1675, 1134, 1695, 1156]
      |       Floating		      off
      |       Location		      [784, 486, 1108, 725]
      |       Open		      off
      |       NumInputPorts	      "1"
      |       ZoomMode		      "yonly"
      |       List {
      | 	ListType		AxesTitles
      | 	axes1			"%<SignalLabel>"
      |       }
      |       TimeRange		      "0.25"
      |       YMin		      "-1"
      |       YMax		      "1"
      |       SaveName		      "ScopeData1"
      |       DataFormat	      "StructureWithTime"
      |       LimitDataPoints	      off
      |       SampleTime	      "0"
      |     }
      |     Block {
      |       BlockType		      Reference
      |       Name		      "Mean1"
      |       Ports		      [1, 1]
      |       Position		      [1175, 1269, 1205, 1301]
      |       DialogController	      "POWERSYS.PowerSysDialog"
      |       FontName		      "Verdana"
      |       FontSize		      11
      |       SourceBlock	      "powerlib_extras/Discrete\nMeasurements/Discrete \nMean value"
      |       SourceType	      "Discrete Mean value"
      |       ShowPortLabels	      "FromPortIcon"
      |       SystemSampleTime	      "-1"
      |       FunctionWithSeparateData off
      |       RTWMemSecFuncInitTerm   "Inherit from model"
      |       RTWMemSecFuncExecute    "Inherit from model"
      |       RTWMemSecDataConstants  "Inherit from model"
      |       RTWMemSecDataInternal   "Inherit from model"
      |       RTWMemSecDataParameters "Inherit from model"
      |       Freq		      "60"
      |       Vinit		      "0"
      |       Ts		      "50e-6"
      |     }
      |     Block {
      |       BlockType		      Reference
      |       Name		      "Mean10"
      |       Ports		      [1, 1]
      |       Position		      [1660, 107, 1680, 133]
      |       DialogController	      "POWERSYS.PowerSysDialog"
      |       FontName		      "Verdana"
      |       FontSize		      11
      |       SourceBlock	      "powerlib_extras/Discrete\nMeasurements/Discrete \nMean value"
      |       SourceType	      "Discrete Mean value"
      |       ShowPortLabels	      "FromPortIcon"
      |       SystemSampleTime	      "-1"
      |       FunctionWithSeparateData off
      |       RTWMemSecFuncInitTerm   "Inherit from model"
      |       RTWMemSecFuncExecute    "Inherit from model"
      |       RTWMemSecDataConstants  "Inherit from model"
      |       RTWMemSecDataInternal   "Inherit from model"
      |       RTWMemSecDataParameters "Inherit from model"
      |       Freq		      "60"
      |       Vinit		      "0"
      |       Ts		      "50e-6"
      |     }
      |     Block {
      |       BlockType		      Reference
      |       Name		      "Mean2"
      |       Ports		      [1, 1]
      |       Position		      [1590, 1117, 1610, 1143]
      |       DialogController	      "POWERSYS.PowerSysDialog"
      |       FontName		      "Verdana"
      |       FontSize		      11
      |       SourceBlock	      "powerlib_extras/Discrete\nMeasurements/Discrete \nMean value"
      |       SourceType	      "Discrete Mean value"
      |       ShowPortLabels	      "FromPortIcon"
      |       SystemSampleTime	      "-1"
      |       FunctionWithSeparateData off
      |       RTWMemSecFuncInitTerm   "Inherit from model"
      |       RTWMemSecFuncExecute    "Inherit from model"
      |       RTWMemSecDataConstants  "Inherit from model"
      |       RTWMemSecDataInternal   "Inherit from model"
      |       RTWMemSecDataParameters "Inherit from model"
      |       Freq		      "60"
      |       Vinit		      "0"
      |       Ts		      "50e-6"
      |     }
      |     Block {
      |       BlockType		      Reference
      |       Name		      "Mean3"
      |       Ports		      [1, 1]
      |       Position		      [305, 654, 335, 686]
      |       DialogController	      "POWERSYS.PowerSysDialog"
      |       FontName		      "Verdana"
      |       FontSize		      11
      |       SourceBlock	      "powerlib_extras/Discrete\nMeasurements/Discrete \nMean value"
      |       SourceType	      "Discrete Mean value"
      |       ShowPortLabels	      "FromPortIcon"
      |       SystemSampleTime	      "-1"
      |       FunctionWithSeparateData off
      |       RTWMemSecFuncInitTerm   "Inherit from model"
      |       RTWMemSecFuncExecute    "Inherit from model"
      |       RTWMemSecDataConstants  "Inherit from model"
      |       RTWMemSecDataInternal   "Inherit from model"
      |       RTWMemSecDataParameters "Inherit from model"
      |       Freq		      "60"
      |       Vinit		      "0"
      |       Ts		      "50e-6"
      |     }
      |     Block {
      |       BlockType		      Reference
      |       Name		      "Mean4"
      |       Ports		      [1, 1]
      |       Position		      [720, 502, 740, 528]
      |       DialogController	      "POWERSYS.PowerSysDialog"
      |       FontName		      "Verdana"
      |       FontSize		      11
      |       SourceBlock	      "powerlib_extras/Discrete\nMeasurements/Discrete \nMean value"
      |       SourceType	      "Discrete Mean value"
      |       ShowPortLabels	      "FromPortIcon"
      |       SystemSampleTime	      "-1"
      |       FunctionWithSeparateData off
      |       RTWMemSecFuncInitTerm   "Inherit from model"
      |       RTWMemSecFuncExecute    "Inherit from model"
      |       RTWMemSecDataConstants  "Inherit from model"
      |       RTWMemSecDataInternal   "Inherit from model"
      |       RTWMemSecDataParameters "Inherit from model"
      |       Freq		      "60"
      |       Vinit		      "0"
      |       Ts		      "50e-6"
      |     }
      |     Block {
      |       BlockType		      Reference
      |       Name		      "Mean5"
      |       Ports		      [1, 1]
      |       Position		      [305, 1219, 335, 1251]
      |       DialogController	      "POWERSYS.PowerSysDialog"
      |       FontName		      "Verdana"
      |       FontSize		      11
      |       SourceBlock	      "powerlib_extras/Discrete\nMeasurements/Discrete \nMean value"
      |       SourceType	      "Discrete Mean value"
      |       ShowPortLabels	      "FromPortIcon"
      |       SystemSampleTime	      "-1"
      |       FunctionWithSeparateData off
      |       RTWMemSecFuncInitTerm   "Inherit from model"
      |       RTWMemSecFuncExecute    "Inherit from model"
      |       RTWMemSecDataConstants  "Inherit from model"
      |       RTWMemSecDataInternal   "Inherit from model"
      |       RTWMemSecDataParameters "Inherit from model"
      |       Freq		      "60"
      |       Vinit		      "0"
      |       Ts		      "50e-6"
      |     }
      |     Block {
      |       BlockType		      Reference
      |       Name		      "Mean6"
      |       Ports		      [1, 1]
      |       Position		      [285, 304, 315, 336]
      |       DialogController	      "POWERSYS.PowerSysDialog"
      |       FontName		      "Verdana"
      |       FontSize		      11
      |       SourceBlock	      "powerlib_extras/Discrete\nMeasurements/Discrete \nMean value"
      |       SourceType	      "Discrete Mean value"
      |       ShowPortLabels	      "FromPortIcon"
      |       SystemSampleTime	      "-1"
      |       FunctionWithSeparateData off
      |       RTWMemSecFuncInitTerm   "Inherit from model"
      |       RTWMemSecFuncExecute    "Inherit from model"
      |       RTWMemSecDataConstants  "Inherit from model"
      |       RTWMemSecDataInternal   "Inherit from model"
      |       RTWMemSecDataParameters "Inherit from model"
      |       Freq		      "60"
      |       Vinit		      "0"
      |       Ts		      "50e-6"
      |     }
      |     Block {
      |       BlockType		      Reference
      |       Name		      "Mean7"
      |       Ports		      [1, 1]
      |       Position		      [700, 152, 720, 178]
      |       DialogController	      "POWERSYS.PowerSysDialog"
      |       FontName		      "Verdana"
      |       FontSize		      11
      |       SourceBlock	      "powerlib_extras/Discrete\nMeasurements/Discrete \nMean value"
      |       SourceType	      "Discrete Mean value"
      |       ShowPortLabels	      "FromPortIcon"
      |       SystemSampleTime	      "-1"
      |       FunctionWithSeparateData off
      |       RTWMemSecFuncInitTerm   "Inherit from model"
      |       RTWMemSecFuncExecute    "Inherit from model"
      |       RTWMemSecDataConstants  "Inherit from model"
      |       RTWMemSecDataInternal   "Inherit from model"
      |       RTWMemSecDataParameters "Inherit from model"
      |       Freq		      "60"
      |       Vinit		      "0"
      |       Ts		      "50e-6"
      |     }
      |     Block {
      |       BlockType		      Reference
      |       Name		      "Mean8"
      |       Ports		      [1, 1]
      |       Position		      [720, 1067, 740, 1093]
      |       DialogController	      "POWERSYS.PowerSysDialog"
      |       FontName		      "Verdana"
      |       FontSize		      11
      |       SourceBlock	      "powerlib_extras/Discrete\nMeasurements/Discrete \nMean value"
      |       SourceType	      "Discrete Mean value"
      |       ShowPortLabels	      "FromPortIcon"
      |       SystemSampleTime	      "-1"
      |       FunctionWithSeparateData off
      |       RTWMemSecFuncInitTerm   "Inherit from model"
      |       RTWMemSecFuncExecute    "Inherit from model"
      |       RTWMemSecDataConstants  "Inherit from model"
      |       RTWMemSecDataInternal   "Inherit from model"
      |       RTWMemSecDataParameters "Inherit from model"
      |       Freq		      "60"
      |       Vinit		      "0"
      |       Ts		      "50e-6"
      |     }
      |     Block {
      |       BlockType		      Reference
      |       Name		      "Mean9"
      |       Ports		      [1, 1]
      |       Position		      [1245, 259, 1275, 291]
      |       DialogController	      "POWERSYS.PowerSysDialog"
      |       FontName		      "Verdana"
      |       FontSize		      11
      |       SourceBlock	      "powerlib_extras/Discrete\nMeasurements/Discrete \nMean value"
      |       SourceType	      "Discrete Mean value"
      |       ShowPortLabels	      "FromPortIcon"
      |       SystemSampleTime	      "-1"
      |       FunctionWithSeparateData off
      |       RTWMemSecFuncInitTerm   "Inherit from model"
      |       RTWMemSecFuncExecute    "Inherit from model"
      |       RTWMemSecDataConstants  "Inherit from model"
      |       RTWMemSecDataInternal   "Inherit from model"
      |       RTWMemSecDataParameters "Inherit from model"
      |       Freq		      "60"
      |       Vinit		      "0"
      |       Ts		      "50e-6"
      |     }
      |     Block {
      |       BlockType		      Mux
      |       Name		      "Mux1"
      |       Ports		      [3, 1]
      |       Position		      [1246, 1305, 1284, 1310]
      |       BlockRotation	      270
      |       BlockMirror	      on
      |       NamePlacement	      "alternate"
      |       ShowName		      off
      |       Inputs		      "3"
      |       DisplayOption	      "bar"
      |     }
      |     Block {
      |       BlockType		      Mux
      |       Name		      "Mux10"
      |       Ports		      [3, 1]
      |       Position		      [376, 690, 414, 695]
      |       BlockRotation	      270
      |       BlockMirror	      on
      |       NamePlacement	      "alternate"
      |       ShowName		      off
      |       Inputs		      "3"
      |       DisplayOption	      "bar"
      |     }
      |     Block {
      |       BlockType		      Mux
      |       Name		      "Mux11"
      |       Ports		      [3, 1]
      |       Position		      [360, 646, 365, 684]
      |       BlockMirror	      on
      |       NamePlacement	      "alternate"
      |       ShowName		      off
      |       Inputs		      "3"
      |       DisplayOption	      "bar"
      |     }
      |     Block {
      |       BlockType		      Mux
      |       Name		      "Mux12"
      |       Ports		      [3, 1]
      |       Position		      [210, 631, 215, 669]
      |       BlockMirror	      on
      |       NamePlacement	      "alternate"
      |       ShowName		      off
      |       Inputs		      "3"
      |       DisplayOption	      "bar"
      |     }
      |     Block {
      |       BlockType		      Mux
      |       Name		      "Mux13"
      |       Ports		      [3, 1]
      |       Position		      [120, 621, 125, 659]
      |       BlockMirror	      on
      |       NamePlacement	      "alternate"
      |       ShowName		      off
      |       Inputs		      "3"
      |       DisplayOption	      "bar"
      |     }
      |     Block {
      |       BlockType		      Mux
      |       Name		      "Mux14"
      |       Ports		      [3, 1]
      |       Position		      [120, 666, 125, 704]
      |       BlockMirror	      on
      |       NamePlacement	      "alternate"
      |       ShowName		      off
      |       Inputs		      "3"
      |       DisplayOption	      "bar"
      |     }
      |     Block {
      |       BlockType		      Mux
      |       Name		      "Mux15"
      |       Ports		      [3, 1]
      |       Position		      [516, 470, 554, 475]
      |       BlockRotation	      270
      |       ShowName		      off
      |       Inputs		      "3"
      |       DisplayOption	      "bar"
      |     }
      |     Block {
      |       BlockType		      Mux
      |       Name		      "Mux16"
      |       Ports		      [3, 1]
      |       Position		      [380, 461, 385, 499]
      |       ShowName		      off
      |       Inputs		      "3"
      |       DisplayOption	      "bar"
      |     }
      |     Block {
      |       BlockType		      Mux
      |       Name		      "Mux17"
      |       Ports		      [3, 1]
      |       Position		      [675, 640, 680, 680]
      |       ShowName		      off
      |       Inputs		      "3"
      |       DisplayOption	      "bar"
      |     }
      |     Block {
      |       BlockType		      Mux
      |       Name		      "Mux18"
      |       Ports		      [3, 1]
      |       Position		      [360, 601, 365, 639]
      |       BlockMirror	      on
      |       NamePlacement	      "alternate"
      |       ShowName		      off
      |       Inputs		      "3"
      |       DisplayOption	      "bar"
      |     }
      |     Block {
      |       BlockType		      Mux
      |       Name		      "Mux19"
      |       Ports		      [3, 1]
      |       Position		      [356, 340, 394, 345]
      |       BlockRotation	      270
      |       BlockMirror	      on
      |       NamePlacement	      "alternate"
      |       ShowName		      off
      |       Inputs		      "3"
      |       DisplayOption	      "bar"
      |     }
      |     Block {
      |       BlockType		      Mux
      |       Name		      "Mux2"
      |       Ports		      [3, 1]
      |       Position		      [1230, 1261, 1235, 1299]
      |       BlockMirror	      on
      |       NamePlacement	      "alternate"
      |       ShowName		      off
      |       Inputs		      "3"
      |       DisplayOption	      "bar"
      |     }
      |     Block {
      |       BlockType		      Mux
      |       Name		      "Mux20"
      |       Ports		      [3, 1]
      |       Position		      [340, 296, 345, 334]
      |       BlockMirror	      on
      |       NamePlacement	      "alternate"
      |       ShowName		      off
      |       Inputs		      "3"
      |       DisplayOption	      "bar"
      |     }
      |     Block {
      |       BlockType		      Mux
      |       Name		      "Mux21"
      |       Ports		      [3, 1]
      |       Position		      [190, 281, 195, 319]
      |       BlockMirror	      on
      |       NamePlacement	      "alternate"
      |       ShowName		      off
      |       Inputs		      "3"
      |       DisplayOption	      "bar"
      |     }
      |     Block {
      |       BlockType		      Mux
      |       Name		      "Mux22"
      |       Ports		      [3, 1]
      |       Position		      [100, 271, 105, 309]
      |       BlockMirror	      on
      |       NamePlacement	      "alternate"
      |       ShowName		      off
      |       Inputs		      "3"
      |       DisplayOption	      "bar"
      |     }
      |     Block {
      |       BlockType		      Mux
      |       Name		      "Mux23"
      |       Ports		      [3, 1]
      |       Position		      [100, 316, 105, 354]
      |       BlockMirror	      on
      |       NamePlacement	      "alternate"
      |       ShowName		      off
      |       Inputs		      "3"
      |       DisplayOption	      "bar"
      |     }
      |     Block {
      |       BlockType		      Mux
      |       Name		      "Mux24"
      |       Ports		      [3, 1]
      |       Position		      [496, 120, 534, 125]
      |       BlockRotation	      270
      |       ShowName		      off
      |       Inputs		      "3"
      |       DisplayOption	      "bar"
      |     }
      |     Block {
      |       BlockType		      Mux
      |       Name		      "Mux25"
      |       Ports		      [3, 1]
      |       Position		      [360, 111, 365, 149]
      |       ShowName		      off
      |       Inputs		      "3"
      |       DisplayOption	      "bar"
      |     }
      |     Block {
      |       BlockType		      Mux
      |       Name		      "Mux26"
      |       Ports		      [3, 1]
      |       Position		      [655, 290, 660, 330]
      |       ShowName		      off
      |       Inputs		      "3"
      |       DisplayOption	      "bar"
      |     }
      |     Block {
      |       BlockType		      Mux
      |       Name		      "Mux27"
      |       Ports		      [3, 1]
      |       Position		      [340, 251, 345, 289]
      |       BlockMirror	      on
      |       NamePlacement	      "alternate"
      |       ShowName		      off
      |       Inputs		      "3"
      |       DisplayOption	      "bar"
      |     }
      |     Block {
      |       BlockType		      Mux
      |       Name		      "Mux28"
      |       Ports		      [3, 1]
      |       Position		      [1316, 295, 1354, 300]
      |       BlockRotation	      270
      |       BlockMirror	      on
      |       NamePlacement	      "alternate"
      |       ShowName		      off
      |       Inputs		      "3"
      |       DisplayOption	      "bar"
      |     }
      |     Block {
      |       BlockType		      Mux
      |       Name		      "Mux29"
      |       Ports		      [3, 1]
      |       Position		      [1300, 251, 1305, 289]
      |       BlockMirror	      on
      |       NamePlacement	      "alternate"
      |       ShowName		      off
      |       Inputs		      "3"
      |       DisplayOption	      "bar"
      |     }
      |     Block {
      |       BlockType		      Mux
      |       Name		      "Mux3"
      |       Ports		      [3, 1]
      |       Position		      [1080, 1246, 1085, 1284]
      |       BlockMirror	      on
      |       NamePlacement	      "alternate"
      |       ShowName		      off
      |       Inputs		      "3"
      |       DisplayOption	      "bar"
      |     }
      |     Block {
      |       BlockType		      Mux
      |       Name		      "Mux30"
      |       Ports		      [3, 1]
      |       Position		      [1150, 236, 1155, 274]
      |       BlockMirror	      on
      |       NamePlacement	      "alternate"
      |       ShowName		      off
      |       Inputs		      "3"
      |       DisplayOption	      "bar"
      |     }
      |     Block {
      |       BlockType		      Mux
      |       Name		      "Mux31"
      |       Ports		      [3, 1]
      |       Position		      [1060, 226, 1065, 264]
      |       BlockMirror	      on
      |       NamePlacement	      "alternate"
      |       ShowName		      off
      |       Inputs		      "3"
      |       DisplayOption	      "bar"
      |     }
      |     Block {
      |       BlockType		      Mux
      |       Name		      "Mux32"
      |       Ports		      [3, 1]
      |       Position		      [1060, 271, 1065, 309]
      |       BlockMirror	      on
      |       NamePlacement	      "alternate"
      |       ShowName		      off
      |       Inputs		      "3"
      |       DisplayOption	      "bar"
      |     }
      |     Block {
      |       BlockType		      Mux
      |       Name		      "Mux33"
      |       Ports		      [3, 1]
      |       Position		      [376, 1255, 414, 1260]
      |       BlockRotation	      270
      |       BlockMirror	      on
      |       NamePlacement	      "alternate"
      |       ShowName		      off
      |       Inputs		      "3"
      |       DisplayOption	      "bar"
      |     }
      |     Block {
      |       BlockType		      Mux
      |       Name		      "Mux34"
      |       Ports		      [3, 1]
      |       Position		      [360, 1211, 365, 1249]
      |       BlockMirror	      on
      |       NamePlacement	      "alternate"
      |       ShowName		      off
      |       Inputs		      "3"
      |       DisplayOption	      "bar"
      |     }
      |     Block {
      |       BlockType		      Mux
      |       Name		      "Mux35"
      |       Ports		      [3, 1]
      |       Position		      [210, 1196, 215, 1234]
      |       BlockMirror	      on
      |       NamePlacement	      "alternate"
      |       ShowName		      off
      |       Inputs		      "3"
      |       DisplayOption	      "bar"
      |     }
      |     Block {
      |       BlockType		      Mux
      |       Name		      "Mux36"
      |       Ports		      [3, 1]
      |       Position		      [120, 1186, 125, 1224]
      |       BlockMirror	      on
      |       NamePlacement	      "alternate"
      |       ShowName		      off
      |       Inputs		      "3"
      |       DisplayOption	      "bar"
      |     }
      |     Block {
      |       BlockType		      Mux
      |       Name		      "Mux37"
      |       Ports		      [3, 1]
      |       Position		      [120, 1231, 125, 1269]
      |       BlockMirror	      on
      |       NamePlacement	      "alternate"
      |       ShowName		      off
      |       Inputs		      "3"
      |       DisplayOption	      "bar"
      |     }
      |     Block {
      |       BlockType		      Mux
      |       Name		      "Mux38"
      |       Ports		      [3, 1]
      |       Position		      [516, 1035, 554, 1040]
      |       BlockRotation	      270
      |       ShowName		      off
      |       Inputs		      "3"
      |       DisplayOption	      "bar"
      |     }
      |     Block {
      |       BlockType		      Mux
      |       Name		      "Mux39"
      |       Ports		      [3, 1]
      |       Position		      [380, 1026, 385, 1064]
      |       ShowName		      off
      |       Inputs		      "3"
      |       DisplayOption	      "bar"
      |     }
      |     Block {
      |       BlockType		      Mux
      |       Name		      "Mux4"
      |       Ports		      [3, 1]
      |       Position		      [990, 1236, 995, 1274]
      |       BlockMirror	      on
      |       NamePlacement	      "alternate"
      |       ShowName		      off
      |       Inputs		      "3"
      |       DisplayOption	      "bar"
      |     }
      |     Block {
      |       BlockType		      Mux
      |       Name		      "Mux40"
      |       Ports		      [3, 1]
      |       Position		      [675, 1205, 680, 1245]
      |       ShowName		      off
      |       Inputs		      "3"
      |       DisplayOption	      "bar"
      |     }
      |     Block {
      |       BlockType		      Mux
      |       Name		      "Mux41"
      |       Ports		      [3, 1]
      |       Position		      [1456, 75, 1494, 80]
      |       BlockRotation	      270
      |       ShowName		      off
      |       Inputs		      "3"
      |       DisplayOption	      "bar"
      |     }
      |     Block {
      |       BlockType		      Mux
      |       Name		      "Mux42"
      |       Ports		      [3, 1]
      |       Position		      [1320, 66, 1325, 104]
      |       ShowName		      off
      |       Inputs		      "3"
      |       DisplayOption	      "bar"
      |     }
      |     Block {
      |       BlockType		      Mux
      |       Name		      "Mux43"
      |       Ports		      [3, 1]
      |       Position		      [360, 1166, 365, 1204]
      |       BlockMirror	      on
      |       NamePlacement	      "alternate"
      |       ShowName		      off
      |       Inputs		      "3"
      |       DisplayOption	      "bar"
      |     }
      |     Block {
      |       BlockType		      Mux
      |       Name		      "Mux44"
      |       Ports		      [3, 1]
      |       Position		      [1615, 245, 1620, 285]
      |       ShowName		      off
      |       Inputs		      "3"
      |       DisplayOption	      "bar"
      |     }
      |     Block {
      |       BlockType		      Mux
      |       Name		      "Mux45"
      |       Ports		      [3, 1]
      |       Position		      [1300, 206, 1305, 244]
      |       BlockMirror	      on
      |       NamePlacement	      "alternate"
      |       ShowName		      off
      |       Inputs		      "3"
      |       DisplayOption	      "bar"
      |     }
      |     Block {
      |       BlockType		      Mux
      |       Name		      "Mux5"
      |       Ports		      [3, 1]
      |       Position		      [990, 1281, 995, 1319]
      |       BlockMirror	      on
      |       NamePlacement	      "alternate"
      |       ShowName		      off
      |       Inputs		      "3"
      |       DisplayOption	      "bar"
      |     }
      |     Block {
      |       BlockType		      Mux
      |       Name		      "Mux6"
      |       Ports		      [3, 1]
      |       Position		      [1386, 1085, 1424, 1090]
      |       BlockRotation	      270
      |       ShowName		      off
      |       Inputs		      "3"
      |       DisplayOption	      "bar"
      |     }
      |     Block {
      |       BlockType		      Mux
      |       Name		      "Mux7"
      |       Ports		      [3, 1]
      |       Position		      [1250, 1076, 1255, 1114]
      |       ShowName		      off
      |       Inputs		      "3"
      |       DisplayOption	      "bar"
      |     }
      |     Block {
      |       BlockType		      Mux
      |       Name		      "Mux8"
      |       Ports		      [3, 1]
      |       Position		      [1545, 1255, 1550, 1295]
      |       ShowName		      off
      |       Inputs		      "3"
      |       DisplayOption	      "bar"
      |     }
      |     Block {
      |       BlockType		      Mux
      |       Name		      "Mux9"
      |       Ports		      [3, 1]
      |       Position		      [1230, 1216, 1235, 1254]
      |       BlockMirror	      on
      |       NamePlacement	      "alternate"
      |       ShowName		      off
      |       Inputs		      "3"
      |       DisplayOption	      "bar"
      |     }
      |     Block {
      |       BlockType		      SubSystem
      |       Name		      "PF1"
      |       Ports		      [1, 1]
      |       Position		      [1175, 1317, 1210, 1343]
      |       BlockMirror	      on
      |       NamePlacement	      "alternate"
      |       PermitHierarchicalResolution "ExplicitOnly"
      |       MinAlgLoopOccurrences   off
      |       PropExecContextOutsideSubsystem off
      |       RTWSystemCode	      "Auto"
      |       FunctionWithSeparateData off
      |       Opaque		      off
      |       Array {
      | 	Type			"Handle"
      | 	Dimension		0
      | 	PropName		"AvailSigsLoadSave"
      |       }
      |       RequestExecContextInheritance off
      |       MaskHideContents	      off
      |       MaskType		      "Stateflow"
      |       MaskDescription	      "Embedded MATLAB block"
      |       MaskDisplay	      "disp('fcn');"
      |       MaskSelfModifiable      on
      |       MaskIconFrame	      on
      |       MaskIconOpaque	      off
      |       MaskIconRotate	      "none"
      |       MaskPortRotate	      "default"
      |       MaskIconUnits	      "autoscale"
      |       System {
      | 	Name			"PF1"
      | 	Location		[257, 457, 812, 717]
      | 	Open			off
      | 	ModelBrowserVisibility	off
      | 	ModelBrowserWidth	200
      | 	ScreenColor		"white"
      | 	PaperOrientation	"landscape"
      | 	PaperPositionMode	"auto"
      | 	PaperType		"usletter"
      | 	PaperUnits		"inches"
      | 	TiledPaperMargins	[0.500000, 0.500000, 0.500000, 0.500000]
      | 	TiledPageScale		1
      | 	ShowPageBoundaries	off
      | 	ZoomFactor		"100"
      | 	Block {
      | 	  BlockType		  Inport
      | 	  Name			  "u"
      | 	  Position		  [20, 101, 40, 119]
      | 	  IconDisplay		  "Port number"
      | 	  OutDataType		  "sfix(16)"
      | 	  OutScaling		  "2^0"
      | 	}
      | 	Block {
      | 	  BlockType		  Demux
      | 	  Name			  " Demux "
      | 	  Ports			  [1, 1]
      | 	  Position		  [270, 160, 320, 200]
      | 	  Outputs		  "1"
      | 	}
      | 	Block {
      | 	  BlockType		  "S-Function"
      | 	  Name			  " SFunction "
      | 	  Tag			  "Stateflow S-Function final_4 1"
      | 	  Ports			  [1, 2]
      | 	  Position		  [180, 100, 230, 160]
      | 	  FunctionName		  "sf_sfun"
      | 	  PortCounts		  "[1 2]"
      | 	  EnableBusSupport	  on
      | 	  Port {
      | 	    PortNumber		    2
      | 	    Name		    "y"
      | 	    RTWStorageClass	    "Auto"
      | 	    DataLoggingNameMode	    "SignalName"
      | 	  }
      | 	}
      | 	Block {
      | 	  BlockType		  Terminator
      | 	  Name			  " Terminator "
      | 	  Position		  [460, 171, 480, 189]
      | 	}
      | 	Block {
      | 	  BlockType		  Outport
      | 	  Name			  "y"
      | 	  Position		  [460, 101, 480, 119]
      | 	  IconDisplay		  "Port number"
      | 	  OutDataType		  "sfix(16)"
      | 	  OutScaling		  "2^0"
      | 	}
      | 	Line {
      | 	  SrcBlock		  " SFunction "
      | 	  SrcPort		  1
      | 	  DstBlock		  " Demux "
      | 	  DstPort		  1
      | 	}
      | 	Line {
      | 	  SrcBlock		  "u"
      | 	  SrcPort		  1
      | 	  DstBlock		  " SFunction "
      | 	  DstPort		  1
      | 	}
      | 	Line {
      | 	  Name			  "y"
      | 	  Labels		  [0, 0]
      | 	  SrcBlock		  " SFunction "
      | 	  SrcPort		  2
      | 	  DstBlock		  "y"
      | 	  DstPort		  1
      | 	}
      | 	Line {
      | 	  SrcBlock		  " Demux "
      | 	  SrcPort		  1
      | 	  DstBlock		  " Terminator "
      | 	  DstPort		  1
      | 	}
      |       }
      |     }
      |     Block {
      |       BlockType		      SubSystem
      |       Name		      "PF10"
      |       Ports		      [1, 1]
      |       Position		      [285, 352, 320, 378]
      |       BlockMirror	      on
      |       NamePlacement	      "alternate"
      |       PermitHierarchicalResolution "ExplicitOnly"
      |       MinAlgLoopOccurrences   off
      |       PropExecContextOutsideSubsystem off
      |       RTWSystemCode	      "Auto"
      |       FunctionWithSeparateData off
      |       Opaque		      off
      |       Array {
      | 	Type			"Handle"
      | 	Dimension		0
      | 	PropName		"AvailSigsLoadSave"
      |       }
      |       RequestExecContextInheritance off
      |       MaskHideContents	      off
      |       MaskType		      "Stateflow"
      |       MaskDescription	      "Embedded MATLAB block"
      |       MaskDisplay	      "disp('fcn');"
      |       MaskSelfModifiable      on
      |       MaskIconFrame	      on
      |       MaskIconOpaque	      off
      |       MaskIconRotate	      "none"
      |       MaskPortRotate	      "default"
      |       MaskIconUnits	      "autoscale"
      |       System {
      | 	Name			"PF10"
      | 	Location		[257, 457, 812, 717]
      | 	Open			off
      | 	ModelBrowserVisibility	off
      | 	ModelBrowserWidth	200
      | 	ScreenColor		"white"
      | 	PaperOrientation	"landscape"
      | 	PaperPositionMode	"auto"
      | 	PaperType		"usletter"
      | 	PaperUnits		"inches"
      | 	TiledPaperMargins	[0.500000, 0.500000, 0.500000, 0.500000]
      | 	TiledPageScale		1
      | 	ShowPageBoundaries	off
      | 	ZoomFactor		"100"
      | 	Block {
      | 	  BlockType		  Inport
      | 	  Name			  "u"
      | 	  Position		  [20, 101, 40, 119]
      | 	  IconDisplay		  "Port number"
      | 	  OutDataType		  "sfix(16)"
      | 	  OutScaling		  "2^0"
      | 	}
      | 	Block {
      | 	  BlockType		  Demux
      | 	  Name			  " Demux "
      | 	  Ports			  [1, 1]
      | 	  Position		  [270, 160, 320, 200]
      | 	  Outputs		  "1"
      | 	}
      | 	Block {
      | 	  BlockType		  "S-Function"
      | 	  Name			  " SFunction "
      | 	  Tag			  "Stateflow S-Function final_4 33"
      | 	  Ports			  [1, 2]
      | 	  Position		  [180, 100, 230, 160]
      | 	  FunctionName		  "sf_sfun"
      | 	  PortCounts		  "[1 2]"
      | 	  EnableBusSupport	  on
      | 	  Port {
      | 	    PortNumber		    2
      | 	    Name		    "y"
      | 	    RTWStorageClass	    "Auto"
      | 	    DataLoggingNameMode	    "SignalName"
      | 	  }
      | 	}
      | 	Block {
      | 	  BlockType		  Terminator
      | 	  Name			  " Terminator "
      | 	  Position		  [460, 171, 480, 189]
      | 	}
      | 	Block {
      | 	  BlockType		  Outport
      | 	  Name			  "y"
      | 	  Position		  [460, 101, 480, 119]
      | 	  IconDisplay		  "Port number"
      | 	  OutDataType		  "sfix(16)"
      | 	  OutScaling		  "2^0"
      | 	}
      | 	Line {
      | 	  SrcBlock		  " SFunction "
      | 	  SrcPort		  1
      | 	  DstBlock		  " Demux "
      | 	  DstPort		  1
      | 	}
      | 	Line {
      | 	  SrcBlock		  "u"
      | 	  SrcPort		  1
      | 	  DstBlock		  " SFunction "
      | 	  DstPort		  1
      | 	}
      | 	Line {
      | 	  Name			  "y"
      | 	  Labels		  [0, 0]
      | 	  SrcBlock		  " SFunction "
      | 	  SrcPort		  2
      | 	  DstBlock		  "y"
      | 	  DstPort		  1
      | 	}
      | 	Line {
      | 	  SrcBlock		  " Demux "
      | 	  SrcPort		  1
      | 	  DstBlock		  " Terminator "
      | 	  DstPort		  1
      | 	}
      |       }
      |     }
      |     Block {
      |       BlockType		      SubSystem
      |       Name		      "PF11"
      |       Ports		      [1, 1]
      |       Position		      [305, 1267, 340, 1293]
      |       BlockMirror	      on
      |       NamePlacement	      "alternate"
      |       PermitHierarchicalResolution "ExplicitOnly"
      |       MinAlgLoopOccurrences   off
      |       PropExecContextOutsideSubsystem off
      |       RTWSystemCode	      "Auto"
      |       FunctionWithSeparateData off
      |       Opaque		      off
      |       Array {
      | 	Type			"Handle"
      | 	Dimension		0
      | 	PropName		"AvailSigsLoadSave"
      |       }
      |       RequestExecContextInheritance off
      |       MaskHideContents	      off
      |       MaskType		      "Stateflow"
      |       MaskDescription	      "Embedded MATLAB block"
      |       MaskDisplay	      "disp('fcn');"
      |       MaskSelfModifiable      on
      |       MaskIconFrame	      on
      |       MaskIconOpaque	      off
      |       MaskIconRotate	      "none"
      |       MaskPortRotate	      "default"
      |       MaskIconUnits	      "autoscale"
      |       System {
      | 	Name			"PF11"
      | 	Location		[257, 457, 812, 717]
      | 	Open			off
      | 	ModelBrowserVisibility	off
      | 	ModelBrowserWidth	200
      | 	ScreenColor		"white"
      | 	PaperOrientation	"landscape"
      | 	PaperPositionMode	"auto"
      | 	PaperType		"usletter"
      | 	PaperUnits		"inches"
      | 	TiledPaperMargins	[0.500000, 0.500000, 0.500000, 0.500000]
      | 	TiledPageScale		1
      | 	ShowPageBoundaries	off
      | 	ZoomFactor		"100"
      | 	Block {
      | 	  BlockType		  Inport
      | 	  Name			  "u"
      | 	  Position		  [20, 101, 40, 119]
      | 	  IconDisplay		  "Port number"
      | 	  OutDataType		  "sfix(16)"
      | 	  OutScaling		  "2^0"
      | 	}
      | 	Block {
      | 	  BlockType		  Demux
      | 	  Name			  " Demux "
      | 	  Ports			  [1, 1]
      | 	  Position		  [270, 160, 320, 200]
      | 	  Outputs		  "1"
      | 	}
      | 	Block {
      | 	  BlockType		  "S-Function"
      | 	  Name			  " SFunction "
      | 	  Tag			  "Stateflow S-Function final_4 17"
      | 	  Ports			  [1, 2]
      | 	  Position		  [180, 100, 230, 160]
      | 	  FunctionName		  "sf_sfun"
      | 	  PortCounts		  "[1 2]"
      | 	  EnableBusSupport	  on
      | 	  Port {
      | 	    PortNumber		    2
      | 	    Name		    "y"
      | 	    RTWStorageClass	    "Auto"
      | 	    DataLoggingNameMode	    "SignalName"
      | 	  }
      | 	}
      | 	Block {
      | 	  BlockType		  Terminator
      | 	  Name			  " Terminator "
      | 	  Position		  [460, 171, 480, 189]
      | 	}
      | 	Block {
      | 	  BlockType		  Outport
      | 	  Name			  "y"
      | 	  Position		  [460, 101, 480, 119]
      | 	  IconDisplay		  "Port number"
      | 	  OutDataType		  "sfix(16)"
      | 	  OutScaling		  "2^0"
      | 	}
      | 	Line {
      | 	  SrcBlock		  " SFunction "
      | 	  SrcPort		  1
      | 	  DstBlock		  " Demux "
      | 	  DstPort		  1
      | 	}
      | 	Line {
      | 	  SrcBlock		  "u"
      | 	  SrcPort		  1
      | 	  DstBlock		  " SFunction "
      | 	  DstPort		  1
      | 	}
      | 	Line {
      | 	  Name			  "y"
      | 	  Labels		  [0, 0]
      | 	  SrcBlock		  " SFunction "
      | 	  SrcPort		  2
      | 	  DstBlock		  "y"
      | 	  DstPort		  1
      | 	}
      | 	Line {
      | 	  SrcBlock		  " Demux "
      | 	  SrcPort		  1
      | 	  DstBlock		  " Terminator "
      | 	  DstPort		  1
      | 	}
      |       }
      |     }
      |     Block {
      |       BlockType		      SubSystem
      |       Name		      "PF12"
      |       Ports		      [1, 1]
      |       Position		      [700, 1045, 730, 1065]
      |       BlockMirror	      on
      |       NamePlacement	      "alternate"
      |       PermitHierarchicalResolution "ExplicitOnly"
      |       MinAlgLoopOccurrences   off
      |       PropExecContextOutsideSubsystem off
      |       RTWSystemCode	      "Auto"
      |       FunctionWithSeparateData off
      |       Opaque		      off
      |       Array {
      | 	Type			"Handle"
      | 	Dimension		0
      | 	PropName		"AvailSigsLoadSave"
      |       }
      |       RequestExecContextInheritance off
      |       MaskHideContents	      off
      |       MaskType		      "Stateflow"
      |       MaskDescription	      "Embedded MATLAB block"
      |       MaskDisplay	      "disp('fcn');"
      |       MaskSelfModifiable      on
      |       MaskIconFrame	      on
      |       MaskIconOpaque	      off
      |       MaskIconRotate	      "none"
      |       MaskPortRotate	      "default"
      |       MaskIconUnits	      "autoscale"
      |       System {
      | 	Name			"PF12"
      | 	Location		[257, 457, 812, 717]
      | 	Open			off
      | 	ModelBrowserVisibility	off
      | 	ModelBrowserWidth	200
      | 	ScreenColor		"white"
      | 	PaperOrientation	"landscape"
      | 	PaperPositionMode	"auto"
      | 	PaperType		"usletter"
      | 	PaperUnits		"inches"
      | 	TiledPaperMargins	[0.500000, 0.500000, 0.500000, 0.500000]
      | 	TiledPageScale		1
      | 	ShowPageBoundaries	off
      | 	ZoomFactor		"100"
      | 	Block {
      | 	  BlockType		  Inport
      | 	  Name			  "u"
      | 	  Position		  [20, 101, 40, 119]
      | 	  IconDisplay		  "Port number"
      | 	  OutDataType		  "sfix(16)"
      | 	  OutScaling		  "2^0"
      | 	}
      | 	Block {
      | 	  BlockType		  Demux
      | 	  Name			  " Demux "
      | 	  Ports			  [1, 1]
      | 	  Position		  [270, 160, 320, 200]
      | 	  Outputs		  "1"
      | 	}
      | 	Block {
      | 	  BlockType		  "S-Function"
      | 	  Name			  " SFunction "
      | 	  Tag			  "Stateflow S-Function final_4 18"
      | 	  Ports			  [1, 2]
      | 	  Position		  [180, 100, 230, 160]
      | 	  FunctionName		  "sf_sfun"
      | 	  PortCounts		  "[1 2]"
      | 	  EnableBusSupport	  on
      | 	  Port {
      | 	    PortNumber		    2
      | 	    Name		    "y"
      | 	    RTWStorageClass	    "Auto"
      | 	    DataLoggingNameMode	    "SignalName"
      | 	  }
      | 	}
      | 	Block {
      | 	  BlockType		  Terminator
      | 	  Name			  " Terminator "
      | 	  Position		  [460, 171, 480, 189]
      | 	}
      | 	Block {
      | 	  BlockType		  Outport
      | 	  Name			  "y"
      | 	  Position		  [460, 101, 480, 119]
      | 	  IconDisplay		  "Port number"
      | 	  OutDataType		  "sfix(16)"
      | 	  OutScaling		  "2^0"
      | 	}
      | 	Line {
      | 	  SrcBlock		  " Demux "
      | 	  SrcPort		  1
      | 	  DstBlock		  " Terminator "
      | 	  DstPort		  1
      | 	}
      | 	Line {
      | 	  Name			  "y"
      | 	  Labels		  [0, 0]
      | 	  SrcBlock		  " SFunction "
      | 	  SrcPort		  2
      | 	  DstBlock		  "y"
      | 	  DstPort		  1
      | 	}
      | 	Line {
      | 	  SrcBlock		  "u"
      | 	  SrcPort		  1
      | 	  DstBlock		  " SFunction "
      | 	  DstPort		  1
      | 	}
      | 	Line {
      | 	  SrcBlock		  " SFunction "
      | 	  SrcPort		  1
      | 	  DstBlock		  " Demux "
      | 	  DstPort		  1
      | 	}
      |       }
      |     }
      |     Block {
      |       BlockType		      SubSystem
      |       Name		      "PF14"
      |       Ports		      [1, 1]
      |       Position		      [680, 130, 710, 150]
      |       BlockMirror	      on
      |       NamePlacement	      "alternate"
      |       PermitHierarchicalResolution "ExplicitOnly"
      |       MinAlgLoopOccurrences   off
      |       PropExecContextOutsideSubsystem off
      |       RTWSystemCode	      "Auto"
      |       FunctionWithSeparateData off
      |       Opaque		      off
      |       Array {
      | 	Type			"Handle"
      | 	Dimension		0
      | 	PropName		"AvailSigsLoadSave"
      |       }
      |       RequestExecContextInheritance off
      |       MaskHideContents	      off
      |       MaskType		      "Stateflow"
      |       MaskDescription	      "Embedded MATLAB block"
      |       MaskDisplay	      "disp('fcn');"
      |       MaskSelfModifiable      on
      |       MaskIconFrame	      on
      |       MaskIconOpaque	      off
      |       MaskIconRotate	      "none"
      |       MaskPortRotate	      "default"
      |       MaskIconUnits	      "autoscale"
      |       System {
      | 	Name			"PF14"
      | 	Location		[257, 457, 812, 717]
      | 	Open			off
      | 	ModelBrowserVisibility	off
      | 	ModelBrowserWidth	200
      | 	ScreenColor		"white"
      | 	PaperOrientation	"landscape"
      | 	PaperPositionMode	"auto"
      | 	PaperType		"usletter"
      | 	PaperUnits		"inches"
      | 	TiledPaperMargins	[0.500000, 0.500000, 0.500000, 0.500000]
      | 	TiledPageScale		1
      | 	ShowPageBoundaries	off
      | 	ZoomFactor		"100"
      | 	Block {
      | 	  BlockType		  Inport
      | 	  Name			  "u"
      | 	  Position		  [20, 101, 40, 119]
      | 	  IconDisplay		  "Port number"
      | 	  OutDataType		  "sfix(16)"
      | 	  OutScaling		  "2^0"
      | 	}
      | 	Block {
      | 	  BlockType		  Demux
      | 	  Name			  " Demux "
      | 	  Ports			  [1, 1]
      | 	  Position		  [270, 160, 320, 200]
      | 	  Outputs		  "1"
      | 	}
      | 	Block {
      | 	  BlockType		  "S-Function"
      | 	  Name			  " SFunction "
      | 	  Tag			  "Stateflow S-Function final_4 34"
      | 	  Ports			  [1, 2]
      | 	  Position		  [180, 100, 230, 160]
      | 	  FunctionName		  "sf_sfun"
      | 	  PortCounts		  "[1 2]"
      | 	  EnableBusSupport	  on
      | 	  Port {
      | 	    PortNumber		    2
      | 	    Name		    "y"
      | 	    RTWStorageClass	    "Auto"
      | 	    DataLoggingNameMode	    "SignalName"
      | 	  }
      | 	}
      | 	Block {
      | 	  BlockType		  Terminator
      | 	  Name			  " Terminator "
      | 	  Position		  [460, 171, 480, 189]
      | 	}
      | 	Block {
      | 	  BlockType		  Outport
      | 	  Name			  "y"
      | 	  Position		  [460, 101, 480, 119]
      | 	  IconDisplay		  "Port number"
      | 	  OutDataType		  "sfix(16)"
      | 	  OutScaling		  "2^0"
      | 	}
      | 	Line {
      | 	  SrcBlock		  " Demux "
      | 	  SrcPort		  1
      | 	  DstBlock		  " Terminator "
      | 	  DstPort		  1
      | 	}
      | 	Line {
      | 	  Name			  "y"
      | 	  Labels		  [0, 0]
      | 	  SrcBlock		  " SFunction "
      | 	  SrcPort		  2
      | 	  DstBlock		  "y"
      | 	  DstPort		  1
      | 	}
      | 	Line {
      | 	  SrcBlock		  "u"
      | 	  SrcPort		  1
      | 	  DstBlock		  " SFunction "
      | 	  DstPort		  1
      | 	}
      | 	Line {
      | 	  SrcBlock		  " SFunction "
      | 	  SrcPort		  1
      | 	  DstBlock		  " Demux "
      | 	  DstPort		  1
      | 	}
      |       }
      |     }
      |     Block {
      |       BlockType		      Scope
      |       Name		      "PF16"
      |       Ports		      [1]
      |       Position		      [245, 349, 275, 381]
      |       BlockMirror	      on
      |       NamePlacement	      "alternate"
      |       Floating		      off
      |       Location		      [-16, 73, 1264, 790]
      |       Open		      off
      |       NumInputPorts	      "1"
      |       List {
      | 	ListType		AxesTitles
      | 	axes1			"%<SignalLabel>"
      |       }
      |       YMin		      "0.9675"
      |       YMax		      "0.9975"
      |       SaveName		      "ScopeData28"
      |       DataFormat	      "StructureWithTime"
      |       LimitDataPoints	      off
      |       SampleTime	      "0"
      |     }
      |     Block {
      |       BlockType		      SubSystem
      |       Name		      "PF17"
      |       Ports		      [1, 1]
      |       Position		      [1245, 307, 1280, 333]
      |       BlockMirror	      on
      |       NamePlacement	      "alternate"
      |       PermitHierarchicalResolution "ExplicitOnly"
      |       MinAlgLoopOccurrences   off
      |       PropExecContextOutsideSubsystem off
      |       RTWSystemCode	      "Auto"
      |       FunctionWithSeparateData off
      |       Opaque		      off
      |       Array {
      | 	Type			"Handle"
      | 	Dimension		0
      | 	PropName		"AvailSigsLoadSave"
      |       }
      |       RequestExecContextInheritance off
      |       MaskHideContents	      off
      |       MaskType		      "Stateflow"
      |       MaskDescription	      "Embedded MATLAB block"
      |       MaskDisplay	      "disp('fcn');"
      |       MaskSelfModifiable      on
      |       MaskIconFrame	      on
      |       MaskIconOpaque	      off
      |       MaskIconRotate	      "none"
      |       MaskPortRotate	      "default"
      |       MaskIconUnits	      "autoscale"
      |       System {
      | 	Name			"PF17"
      | 	Location		[257, 457, 812, 717]
      | 	Open			off
      | 	ModelBrowserVisibility	off
      | 	ModelBrowserWidth	200
      | 	ScreenColor		"white"
      | 	PaperOrientation	"landscape"
      | 	PaperPositionMode	"auto"
      | 	PaperType		"usletter"
      | 	PaperUnits		"inches"
      | 	TiledPaperMargins	[0.500000, 0.500000, 0.500000, 0.500000]
      | 	TiledPageScale		1
      | 	ShowPageBoundaries	off
      | 	ZoomFactor		"100"
      | 	Block {
      | 	  BlockType		  Inport
      | 	  Name			  "u"
      | 	  Position		  [20, 101, 40, 119]
      | 	  IconDisplay		  "Port number"
      | 	  OutDataType		  "sfix(16)"
      | 	  OutScaling		  "2^0"
      | 	}
      | 	Block {
      | 	  BlockType		  Demux
      | 	  Name			  " Demux "
      | 	  Ports			  [1, 1]
      | 	  Position		  [270, 160, 320, 200]
      | 	  Outputs		  "1"
      | 	}
      | 	Block {
      | 	  BlockType		  "S-Function"
      | 	  Name			  " SFunction "
      | 	  Tag			  "Stateflow S-Function final_4 56"
      | 	  Ports			  [1, 2]
      | 	  Position		  [180, 100, 230, 160]
      | 	  FunctionName		  "sf_sfun"
      | 	  PortCounts		  "[1 2]"
      | 	  EnableBusSupport	  on
      | 	  Port {
      | 	    PortNumber		    2
      | 	    Name		    "y"
      | 	    RTWStorageClass	    "Auto"
      | 	    DataLoggingNameMode	    "SignalName"
      | 	  }
      | 	}
      | 	Block {
      | 	  BlockType		  Terminator
      | 	  Name			  " Terminator "
      | 	  Position		  [460, 171, 480, 189]
      | 	}
      | 	Block {
      | 	  BlockType		  Outport
      | 	  Name			  "y"
      | 	  Position		  [460, 101, 480, 119]
      | 	  IconDisplay		  "Port number"
      | 	  OutDataType		  "sfix(16)"
      | 	  OutScaling		  "2^0"
      | 	}
      | 	Line {
      | 	  SrcBlock		  " SFunction "
      | 	  SrcPort		  1
      | 	  DstBlock		  " Demux "
      | 	  DstPort		  1
      | 	}
      | 	Line {
      | 	  SrcBlock		  "u"
      | 	  SrcPort		  1
      | 	  DstBlock		  " SFunction "
      | 	  DstPort		  1
      | 	}
      | 	Line {
      | 	  Name			  "y"
      | 	  Labels		  [0, 0]
      | 	  SrcBlock		  " SFunction "
      | 	  SrcPort		  2
      | 	  DstBlock		  "y"
      | 	  DstPort		  1
      | 	}
      | 	Line {
      | 	  SrcBlock		  " Demux "
      | 	  SrcPort		  1
      | 	  DstBlock		  " Terminator "
      | 	  DstPort		  1
      | 	}
      |       }
      |     }
      |     Block {
      |       BlockType		      SubSystem
      |       Name		      "PF18"
      |       Ports		      [1, 1]
      |       Position		      [1640, 85, 1670, 105]
      |       BlockMirror	      on
      |       NamePlacement	      "alternate"
      |       PermitHierarchicalResolution "ExplicitOnly"
      |       MinAlgLoopOccurrences   off
      |       PropExecContextOutsideSubsystem off
      |       RTWSystemCode	      "Auto"
      |       FunctionWithSeparateData off
      |       Opaque		      off
      |       Array {
      | 	Type			"Handle"
      | 	Dimension		0
      | 	PropName		"AvailSigsLoadSave"
      |       }
      |       RequestExecContextInheritance off
      |       MaskHideContents	      off
      |       MaskType		      "Stateflow"
      |       MaskDescription	      "Embedded MATLAB block"
      |       MaskDisplay	      "disp('fcn');"
      |       MaskSelfModifiable      on
      |       MaskIconFrame	      on
      |       MaskIconOpaque	      off
      |       MaskIconRotate	      "none"
      |       MaskPortRotate	      "default"
      |       MaskIconUnits	      "autoscale"
      |       System {
      | 	Name			"PF18"
      | 	Location		[257, 457, 812, 717]
      | 	Open			off
      | 	ModelBrowserVisibility	off
      | 	ModelBrowserWidth	200
      | 	ScreenColor		"white"
      | 	PaperOrientation	"landscape"
      | 	PaperPositionMode	"auto"
      | 	PaperType		"usletter"
      | 	PaperUnits		"inches"
      | 	TiledPaperMargins	[0.500000, 0.500000, 0.500000, 0.500000]
      | 	TiledPageScale		1
      | 	ShowPageBoundaries	off
      | 	ZoomFactor		"100"
      | 	Block {
      | 	  BlockType		  Inport
      | 	  Name			  "u"
      | 	  Position		  [20, 101, 40, 119]
      | 	  IconDisplay		  "Port number"
      | 	  OutDataType		  "sfix(16)"
      | 	  OutScaling		  "2^0"
      | 	}
      | 	Block {
      | 	  BlockType		  Demux
      | 	  Name			  " Demux "
      | 	  Ports			  [1, 1]
      | 	  Position		  [270, 160, 320, 200]
      | 	  Outputs		  "1"
      | 	}
      | 	Block {
      | 	  BlockType		  "S-Function"
      | 	  Name			  " SFunction "
      | 	  Tag			  "Stateflow S-Function final_4 57"
      | 	  Ports			  [1, 2]
      | 	  Position		  [180, 100, 230, 160]
      | 	  FunctionName		  "sf_sfun"
      | 	  PortCounts		  "[1 2]"
      | 	  EnableBusSupport	  on
      | 	  Port {
      | 	    PortNumber		    2
      | 	    Name		    "y"
      | 	    RTWStorageClass	    "Auto"
      | 	    DataLoggingNameMode	    "SignalName"
      | 	  }
      | 	}
      | 	Block {
      | 	  BlockType		  Terminator
      | 	  Name			  " Terminator "
      | 	  Position		  [460, 171, 480, 189]
      | 	}
      | 	Block {
      | 	  BlockType		  Outport
      | 	  Name			  "y"
      | 	  Position		  [460, 101, 480, 119]
      | 	  IconDisplay		  "Port number"
      | 	  OutDataType		  "sfix(16)"
      | 	  OutScaling		  "2^0"
      | 	}
      | 	Line {
      | 	  SrcBlock		  " Demux "
      | 	  SrcPort		  1
      | 	  DstBlock		  " Terminator "
      | 	  DstPort		  1
      | 	}
      | 	Line {
      | 	  Name			  "y"
      | 	  Labels		  [0, 0]
      | 	  SrcBlock		  " SFunction "
      | 	  SrcPort		  2
      | 	  DstBlock		  "y"
      | 	  DstPort		  1
      | 	}
      | 	Line {
      | 	  SrcBlock		  "u"
      | 	  SrcPort		  1
      | 	  DstBlock		  " SFunction "
      | 	  DstPort		  1
      | 	}
      | 	Line {
      | 	  SrcBlock		  " SFunction "
      | 	  SrcPort		  1
      | 	  DstBlock		  " Demux "
      | 	  DstPort		  1
      | 	}
      |       }
      |     }
      |     Block {
      |       BlockType		      SubSystem
      |       Name		      "PF2"
      |       Ports		      [1, 1]
      |       Position		      [1570, 1095, 1600, 1115]
      |       BlockMirror	      on
      |       NamePlacement	      "alternate"
      |       PermitHierarchicalResolution "ExplicitOnly"
      |       MinAlgLoopOccurrences   off
      |       PropExecContextOutsideSubsystem off
      |       RTWSystemCode	      "Auto"
      |       FunctionWithSeparateData off
      |       Opaque		      off
      |       Array {
      | 	Type			"Handle"
      | 	Dimension		0
      | 	PropName		"AvailSigsLoadSave"
      |       }
      |       RequestExecContextInheritance off
      |       MaskHideContents	      off
      |       MaskType		      "Stateflow"
      |       MaskDescription	      "Embedded MATLAB block"
      |       MaskDisplay	      "disp('fcn');"
      |       MaskSelfModifiable      on
      |       MaskIconFrame	      on
      |       MaskIconOpaque	      off
      |       MaskIconRotate	      "none"
      |       MaskPortRotate	      "default"
      |       MaskIconUnits	      "autoscale"
      |       System {
      | 	Name			"PF2"
      | 	Location		[257, 457, 812, 717]
      | 	Open			off
      | 	ModelBrowserVisibility	off
      | 	ModelBrowserWidth	200
      | 	ScreenColor		"white"
      | 	PaperOrientation	"landscape"
      | 	PaperPositionMode	"auto"
      | 	PaperType		"usletter"
      | 	PaperUnits		"inches"
      | 	TiledPaperMargins	[0.500000, 0.500000, 0.500000, 0.500000]
      | 	TiledPageScale		1
      | 	ShowPageBoundaries	off
      | 	ZoomFactor		"100"
      | 	Block {
      | 	  BlockType		  Inport
      | 	  Name			  "u"
      | 	  Position		  [20, 101, 40, 119]
      | 	  IconDisplay		  "Port number"
      | 	  OutDataType		  "sfix(16)"
      | 	  OutScaling		  "2^0"
      | 	}
      | 	Block {
      | 	  BlockType		  Demux
      | 	  Name			  " Demux "
      | 	  Ports			  [1, 1]
      | 	  Position		  [270, 160, 320, 200]
      | 	  Outputs		  "1"
      | 	}
      | 	Block {
      | 	  BlockType		  "S-Function"
      | 	  Name			  " SFunction "
      | 	  Tag			  "Stateflow S-Function final_4 2"
      | 	  Ports			  [1, 2]
      | 	  Position		  [180, 100, 230, 160]
      | 	  FunctionName		  "sf_sfun"
      | 	  PortCounts		  "[1 2]"
      | 	  EnableBusSupport	  on
      | 	  Port {
      | 	    PortNumber		    2
      | 	    Name		    "y"
      | 	    RTWStorageClass	    "Auto"
      | 	    DataLoggingNameMode	    "SignalName"
      | 	  }
      | 	}
      | 	Block {
      | 	  BlockType		  Terminator
      | 	  Name			  " Terminator "
      | 	  Position		  [460, 171, 480, 189]
      | 	}
      | 	Block {
      | 	  BlockType		  Outport
      | 	  Name			  "y"
      | 	  Position		  [460, 101, 480, 119]
      | 	  IconDisplay		  "Port number"
      | 	  OutDataType		  "sfix(16)"
      | 	  OutScaling		  "2^0"
      | 	}
      | 	Line {
      | 	  SrcBlock		  " Demux "
      | 	  SrcPort		  1
      | 	  DstBlock		  " Terminator "
      | 	  DstPort		  1
      | 	}
      | 	Line {
      | 	  Name			  "y"
      | 	  Labels		  [0, 0]
      | 	  SrcBlock		  " SFunction "
      | 	  SrcPort		  2
      | 	  DstBlock		  "y"
      | 	  DstPort		  1
      | 	}
      | 	Line {
      | 	  SrcBlock		  "u"
      | 	  SrcPort		  1
      | 	  DstBlock		  " SFunction "
      | 	  DstPort		  1
      | 	}
      | 	Line {
      | 	  SrcBlock		  " SFunction "
      | 	  SrcPort		  1
      | 	  DstBlock		  " Demux "
      | 	  DstPort		  1
      | 	}
      |       }
      |     }
      |     Block {
      |       BlockType		      SubSystem
      |       Name		      "PF6"
      |       Ports		      [1, 1]
      |       Position		      [305, 702, 340, 728]
      |       BlockMirror	      on
      |       NamePlacement	      "alternate"
      |       PermitHierarchicalResolution "ExplicitOnly"
      |       MinAlgLoopOccurrences   off
      |       PropExecContextOutsideSubsystem off
      |       RTWSystemCode	      "Auto"
      |       FunctionWithSeparateData off
      |       Opaque		      off
      |       Array {
      | 	Type			"Handle"
      | 	Dimension		0
      | 	PropName		"AvailSigsLoadSave"
      |       }
      |       RequestExecContextInheritance off
      |       MaskHideContents	      off
      |       MaskType		      "Stateflow"
      |       MaskDescription	      "Embedded MATLAB block"
      |       MaskDisplay	      "disp('fcn');"
      |       MaskSelfModifiable      on
      |       MaskIconFrame	      on
      |       MaskIconOpaque	      off
      |       MaskIconRotate	      "none"
      |       MaskPortRotate	      "default"
      |       MaskIconUnits	      "autoscale"
      |       System {
      | 	Name			"PF6"
      | 	Location		[257, 457, 812, 717]
      | 	Open			off
      | 	ModelBrowserVisibility	off
      | 	ModelBrowserWidth	200
      | 	ScreenColor		"white"
      | 	PaperOrientation	"landscape"
      | 	PaperPositionMode	"auto"
      | 	PaperType		"usletter"
      | 	PaperUnits		"inches"
      | 	TiledPaperMargins	[0.500000, 0.500000, 0.500000, 0.500000]
      | 	TiledPageScale		1
      | 	ShowPageBoundaries	off
      | 	ZoomFactor		"100"
      | 	Block {
      | 	  BlockType		  Inport
      | 	  Name			  "u"
      | 	  Position		  [20, 101, 40, 119]
      | 	  IconDisplay		  "Port number"
      | 	  OutDataType		  "sfix(16)"
      | 	  OutScaling		  "2^0"
      | 	}
      | 	Block {
      | 	  BlockType		  Demux
      | 	  Name			  " Demux "
      | 	  Ports			  [1, 1]
      | 	  Position		  [270, 160, 320, 200]
      | 	  Outputs		  "1"
      | 	}
      | 	Block {
      | 	  BlockType		  "S-Function"
      | 	  Name			  " SFunction "
      | 	  Tag			  "Stateflow S-Function final_4 15"
      | 	  Ports			  [1, 2]
      | 	  Position		  [180, 100, 230, 160]
      | 	  FunctionName		  "sf_sfun"
      | 	  PortCounts		  "[1 2]"
      | 	  EnableBusSupport	  on
      | 	  Port {
      | 	    PortNumber		    2
      | 	    Name		    "y"
      | 	    RTWStorageClass	    "Auto"
      | 	    DataLoggingNameMode	    "SignalName"
      | 	  }
      | 	}
      | 	Block {
      | 	  BlockType		  Terminator
      | 	  Name			  " Terminator "
      | 	  Position		  [460, 171, 480, 189]
      | 	}
      | 	Block {
      | 	  BlockType		  Outport
      | 	  Name			  "y"
      | 	  Position		  [460, 101, 480, 119]
      | 	  IconDisplay		  "Port number"
      | 	  OutDataType		  "sfix(16)"
      | 	  OutScaling		  "2^0"
      | 	}
      | 	Line {
      | 	  SrcBlock		  " SFunction "
      | 	  SrcPort		  1
      | 	  DstBlock		  " Demux "
      | 	  DstPort		  1
      | 	}
      | 	Line {
      | 	  SrcBlock		  "u"
      | 	  SrcPort		  1
      | 	  DstBlock		  " SFunction "
      | 	  DstPort		  1
      | 	}
      | 	Line {
      | 	  Name			  "y"
      | 	  Labels		  [0, 0]
      | 	  SrcBlock		  " SFunction "
      | 	  SrcPort		  2
      | 	  DstBlock		  "y"
      | 	  DstPort		  1
      | 	}
      | 	Line {
      | 	  SrcBlock		  " Demux "
      | 	  SrcPort		  1
      | 	  DstBlock		  " Terminator "
      | 	  DstPort		  1
      | 	}
      |       }
      |     }
      |     Block {
      |       BlockType		      Scope
      |       Name		      "PF8"
      |       Ports		      [1]
      |       Position		      [700, 434, 730, 466]
      |       Floating		      off
      |       Location		      [5, 73, 1285, 790]
      |       Open		      off
      |       NumInputPorts	      "1"
      |       List {
      | 	ListType		AxesTitles
      | 	axes1			"%<SignalLabel>"
      |       }
      |       YMin		      "0.9961"
      |       YMax		      "0.9978"
      |       SaveName		      "ScopeData12"
      |       DataFormat	      "StructureWithTime"
      |       LimitDataPoints	      off
      |       SampleTime	      "0"
      |     }
      |     Block {
      |       BlockType		      Scope
      |       Name		      "PF_1"
      |       Ports		      [1]
      |       Position		      [695, 89, 725, 121]
      |       Floating		      off
      |       Location		      [5, 73, 1285, 790]
      |       Open		      off
      |       NumInputPorts	      "1"
      |       List {
      | 	ListType		AxesTitles
      | 	axes1			"%<SignalLabel>"
      |       }
      |       YMin		      "0.9961"
      |       YMax		      "0.9978"
      |       SaveName		      "ScopeData22"
      |       DataFormat	      "StructureWithTime"
      |       LimitDataPoints	      off
      |       SampleTime	      "0"
      |     }
      |     Block {
      |       BlockType		      SubSystem
      |       Name		      "PF_2"
      |       Ports		      [1, 1]
      |       Position		      [700, 480, 730, 500]
      |       BlockMirror	      on
      |       NamePlacement	      "alternate"
      |       PermitHierarchicalResolution "ExplicitOnly"
      |       MinAlgLoopOccurrences   off
      |       PropExecContextOutsideSubsystem off
      |       RTWSystemCode	      "Auto"
      |       FunctionWithSeparateData off
      |       Opaque		      off
      |       Array {
      | 	Type			"Handle"
      | 	Dimension		0
      | 	PropName		"AvailSigsLoadSave"
      |       }
      |       RequestExecContextInheritance off
      |       MaskHideContents	      off
      |       MaskType		      "Stateflow"
      |       MaskDescription	      "Embedded MATLAB block"
      |       MaskDisplay	      "disp('fcn');"
      |       MaskSelfModifiable      on
      |       MaskIconFrame	      on
      |       MaskIconOpaque	      off
      |       MaskIconRotate	      "none"
      |       MaskPortRotate	      "default"
      |       MaskIconUnits	      "autoscale"
      |       System {
      | 	Name			"PF_2"
      | 	Location		[257, 457, 812, 717]
      | 	Open			off
      | 	ModelBrowserVisibility	off
      | 	ModelBrowserWidth	200
      | 	ScreenColor		"white"
      | 	PaperOrientation	"landscape"
      | 	PaperPositionMode	"auto"
      | 	PaperType		"usletter"
      | 	PaperUnits		"inches"
      | 	TiledPaperMargins	[0.500000, 0.500000, 0.500000, 0.500000]
      | 	TiledPageScale		1
      | 	ShowPageBoundaries	off
      | 	ZoomFactor		"100"
      | 	Block {
      | 	  BlockType		  Inport
      | 	  Name			  "u"
      | 	  Position		  [20, 101, 40, 119]
      | 	  IconDisplay		  "Port number"
      | 	  OutDataType		  "sfix(16)"
      | 	  OutScaling		  "2^0"
      | 	}
      | 	Block {
      | 	  BlockType		  Demux
      | 	  Name			  " Demux "
      | 	  Ports			  [1, 1]
      | 	  Position		  [270, 160, 320, 200]
      | 	  Outputs		  "1"
      | 	}
      | 	Block {
      | 	  BlockType		  "S-Function"
      | 	  Name			  " SFunction "
      | 	  Tag			  "Stateflow S-Function final_4 16"
      | 	  Ports			  [1, 2]
      | 	  Position		  [180, 100, 230, 160]
      | 	  FunctionName		  "sf_sfun"
      | 	  PortCounts		  "[1 2]"
      | 	  EnableBusSupport	  on
      | 	  Port {
      | 	    PortNumber		    2
      | 	    Name		    "y"
      | 	    RTWStorageClass	    "Auto"
      | 	    DataLoggingNameMode	    "SignalName"
      | 	  }
      | 	}
      | 	Block {
      | 	  BlockType		  Terminator
      | 	  Name			  " Terminator "
      | 	  Position		  [460, 171, 480, 189]
      | 	}
      | 	Block {
      | 	  BlockType		  Outport
      | 	  Name			  "y"
      | 	  Position		  [460, 101, 480, 119]
      | 	  IconDisplay		  "Port number"
      | 	  OutDataType		  "sfix(16)"
      | 	  OutScaling		  "2^0"
      | 	}
      | 	Line {
      | 	  SrcBlock		  " Demux "
      | 	  SrcPort		  1
      | 	  DstBlock		  " Terminator "
      | 	  DstPort		  1
      | 	}
      | 	Line {
      | 	  Name			  "y"
      | 	  Labels		  [0, 0]
      | 	  SrcBlock		  " SFunction "
      | 	  SrcPort		  2
      | 	  DstBlock		  "y"
      | 	  DstPort		  1
      | 	}
      | 	Line {
      | 	  SrcBlock		  "u"
      | 	  SrcPort		  1
      | 	  DstBlock		  " SFunction "
      | 	  DstPort		  1
      | 	}
      | 	Line {
      | 	  SrcBlock		  " SFunction "
      | 	  SrcPort		  1
      | 	  DstBlock		  " Demux "
      | 	  DstPort		  1
      | 	}
      |       }
      |     }
      |     Block {
      |       BlockType		      Scope
      |       Name		      "PF_3"
      |       Ports		      [1]
      |       Position		      [700, 989, 730, 1021]
      |       Floating		      off
      |       Location		      [5, 73, 1285, 790]
      |       Open		      off
      |       NumInputPorts	      "1"
      |       List {
      | 	ListType		AxesTitles
      | 	axes1			"%<SignalLabel>"
      |       }
      |       YMin		      "0.9961"
      |       YMax		      "0.9978"
      |       SaveName		      "ScopeData23"
      |       DataFormat	      "StructureWithTime"
      |       LimitDataPoints	      off
      |       SampleTime	      "0"
      |     }
      |     Block {
      |       BlockType		      Scope
      |       Name		      "PF_4"
      |       Ports		      [1]
      |       Position		      [1640, 34, 1670, 66]
      |       Floating		      off
      |       Location		      [5, 73, 1285, 790]
      |       Open		      off
      |       NumInputPorts	      "1"
      |       List {
      | 	ListType		AxesTitles
      | 	axes1			"%<SignalLabel>"
      |       }
      |       YMin		      "0.9961"
      |       YMax		      "0.9978"
      |       SaveName		      "ScopeData45"
      |       DataFormat	      "StructureWithTime"
      |       LimitDataPoints	      off
      |       SampleTime	      "0"
      |     }
      |     Block {
      |       BlockType		      Scope
      |       Name		      "PF_5"
      |       Ports		      [1]
      |       Position		      [1570, 1044, 1600, 1076]
      |       Floating		      off
      |       Location		      [5, 73, 1285, 790]
      |       Open		      off
      |       NumInputPorts	      "1"
      |       List {
      | 	ListType		AxesTitles
      | 	axes1			"%<SignalLabel>"
      |       }
      |       YMin		      "0.9961"
      |       YMax		      "0.9978"
      |       SaveName		      "ScopeData2"
      |       DataFormat	      "StructureWithTime"
      |       LimitDataPoints	      off
      |       SampleTime	      "0"
      |     }
      |     Block {
      |       BlockType		      Scope
      |       Name		      "PF_L2"
      |       Ports		      [1]
      |       Position		      [265, 699, 295, 731]
      |       BlockMirror	      on
      |       NamePlacement	      "alternate"
      |       Floating		      off
      |       Location		      [-16, 73, 1264, 790]
      |       Open		      off
      |       NumInputPorts	      "1"
      |       List {
      | 	ListType		AxesTitles
      | 	axes1			"%<SignalLabel>"
      |       }
      |       YMin		      "0.9675"
      |       YMax		      "0.9975"
      |       SaveName		      "ScopeData13"
      |       DataFormat	      "StructureWithTime"
      |       LimitDataPoints	      off
      |       SampleTime	      "0"
      |     }
      |     Block {
      |       BlockType		      Scope
      |       Name		      "PF_L3"
      |       Ports		      [1]
      |       Position		      [265, 1264, 295, 1296]
      |       BlockMirror	      on
      |       NamePlacement	      "alternate"
      |       Floating		      off
      |       Location		      [-16, 73, 1264, 790]
      |       Open		      off
      |       NumInputPorts	      "1"
      |       List {
      | 	ListType		AxesTitles
      | 	axes1			"%<SignalLabel>"
      |       }
      |       YMin		      "0.9675"
      |       YMax		      "0.9975"
      |       SaveName		      "ScopeData24"
      |       DataFormat	      "StructureWithTime"
      |       LimitDataPoints	      off
      |       SampleTime	      "0"
      |     }
      |     Block {
      |       BlockType		      Scope
      |       Name		      "PF_L4"
      |       Ports		      [1]
      |       Position		      [1205, 304, 1235, 336]
      |       BlockMirror	      on
      |       NamePlacement	      "alternate"
      |       Floating		      off
      |       Location		      [-16, 73, 1264, 790]
      |       Open		      off
      |       NumInputPorts	      "1"
      |       List {
      | 	ListType		AxesTitles
      | 	axes1			"%<SignalLabel>"
      |       }
      |       YMin		      "0.9675"
      |       YMax		      "0.9975"
      |       SaveName		      "ScopeData46"
      |       DataFormat	      "StructureWithTime"
      |       LimitDataPoints	      off
      |       SampleTime	      "0"
      |     }
      |     Block {
      |       BlockType		      Scope
      |       Name		      "PF_L5"
      |       Ports		      [1]
      |       Position		      [1135, 1314, 1165, 1346]
      |       BlockMirror	      on
      |       NamePlacement	      "alternate"
      |       Floating		      off
      |       Location		      [5, 73, 1285, 790]
      |       Open		      off
      |       NumInputPorts	      "1"
      |       List {
      | 	ListType		AxesTitles
      | 	axes1			"%<SignalLabel>"
      |       }
      |       YMin		      "0.9675"
      |       YMax		      "0.9975"
      |       SaveName		      "ScopeData3"
      |       DataFormat	      "StructureWithTime"
      |       LimitDataPoints	      off
      |       SampleTime	      "0"
      |     }
      |     Block {
      |       BlockType		      Reference
      |       Name		      "PQ1"
      |       Ports		      [2, 1]
      |       Position		      [1155, 1225, 1195, 1260]
      |       BlockMirror	      on
      |       NamePlacement	      "alternate"
      |       DialogController	      "POWERSYS.PowerSysDialog"
      |       FontName		      "Verdana"
      |       FontSize		      11
      |       SourceBlock	      "powerlib_extras/Measurements/3-phase \nInstantaneous \nActive & Reactive Power"
      |       SourceType	      "3-phase instantaneous active and reactive power"
      |       ShowPortLabels	      "FromPortIcon"
      |       SystemSampleTime	      "-1"
      |       FunctionWithSeparateData off
      |       RTWMemSecFuncInitTerm   "Inherit from model"
      |       RTWMemSecFuncExecute    "Inherit from model"
      |       RTWMemSecDataConstants  "Inherit from model"
      |       RTWMemSecDataInternal   "Inherit from model"
      |       RTWMemSecDataParameters "Inherit from model"
      |     }
      |     Block {
      |       BlockType		      Reference
      |       Name		      "PQ10"
      |       Ports		      [2, 1]
      |       Position		      [1650, 166, 1675, 199]
      |       NamePlacement	      "alternate"
      |       DialogController	      "POWERSYS.PowerSysDialog"
      |       FontName		      "Verdana"
      |       FontSize		      11
      |       SourceBlock	      "powerlib_extras/Measurements/3-phase \nInstantaneous \nActive & Reactive Power"
      |       SourceType	      "3-phase instantaneous active and reactive power"
      |       ShowPortLabels	      "FromPortIcon"
      |       SystemSampleTime	      "-1"
      |       FunctionWithSeparateData off
      |       RTWMemSecFuncInitTerm   "Inherit from model"
      |       RTWMemSecFuncExecute    "Inherit from model"
      |       RTWMemSecDataConstants  "Inherit from model"
      |       RTWMemSecDataInternal   "Inherit from model"
      |       RTWMemSecDataParameters "Inherit from model"
      |     }
      |     Block {
      |       BlockType		      Reference
